simulink model "simulator_prototype_v2"  (R2021b)
(part 11 of 12)

t7145 = ct{1618};
t7148 = ct{1619};
t7149 = ct{1620};
t7150 = ct{1621};
t7152 = ct{1622};
t7153 = ct{1623};
t7156 = ct{1624};
t7157 = ct{1625};
t7159 = ct{1626};
t7160 = ct{1627};
t7163 = ct{1628};
t7164 = ct{1629};
t7166 = ct{1630};
t7167 = ct{1631};
t7168 = ct{1632};
t7169 = ct{1633};
t7171 = ct{1634};
t7172 = ct{1635};
t7175 = ct{1636};
t7176 = ct{1637};
t7179 = ct{1638};
t7181 = ct{1639};
t7185 = ct{1640};
t7186 = ct{1641};
t7195 = ct{1642};
t7196 = ct{1643};
t7200 = ct{1644};
t7201 = ct{1645};
t7202 = ct{1646};
t7203 = ct{1647};
t7204 = ct{1648};
t7209 = ct{1649};
t721 = ct{1650};
t7211 = ct{1651};
t7212 = ct{1652};
t7219 = ct{1653};
t722 = ct{1654};
t7223 = ct{1655};
t7224 = ct{1656};
t7225 = ct{1657};
t7232 = ct{1658};
t7233 = ct{1659};
t7235 = ct{1660};
t724 = ct{1661};
t7240 = ct{1662};
t7242 = ct{1663};
t7245 = ct{1664};
t7246 = ct{1665};
t7250 = ct{1666};
t7252 = ct{1667};
t7253 = ct{1668};
t7254 = ct{1669};
t7255 = ct{1670};
t7257 = ct{1671};
t7259 = ct{1672};
t7266 = ct{1673};
t7268 = ct{1674};
t7277 = ct{1675};
t7278 = ct{1676};
t7282 = ct{1677};
t7284 = ct{1678};
t7285 = ct{1679};
t7286 = ct{1680};
t7287 = ct{1681};
t7288 = ct{1682};
t7290 = ct{1683};
t7292 = ct{1684};
t7293 = ct{1685};
t7295 = ct{1686};
t7296 = ct{1687};
t7297 = ct{1688};
t7298 = ct{1689};
t7299 = ct{1690};
t7300 = ct{1691};
t7301 = ct{1692};
t7302 = ct{1693};
t7303 = ct{1694};
t7304 = ct{1695};
t7305 = ct{1696};
t7306 = ct{1697};
t7307 = ct{1698};
t7308 = ct{1699};
t7309 = ct{1700};
t7311 = ct{1701};
t7313 = ct{1702};
t7316 = ct{1703};
t7317 = ct{1704};
t7325 = ct{1705};
t7326 = ct{1706};
t7331 = ct{1707};
t7333 = ct{1708};
t7334 = ct{1709};
t7336 = ct{1710};
t7337 = ct{1711};
t7339 = ct{1712};
t7340 = ct{1713};
t7342 = ct{1714};
t7343 = ct{1715};
t7345 = ct{1716};
t7346 = ct{1717};
t7347 = ct{1718};
t7349 = ct{1719};
t7351 = ct{1720};
t7353 = ct{1721};
t7354 = ct{1722};
t7359 = ct{1723};
t7360 = ct{1724};
t7361 = ct{1725};
t7362 = ct{1726};
t7363 = ct{1727};
t7371 = ct{1728};
t7372 = ct{1729};
t7375 = ct{1730};
t7381 = ct{1731};
t7382 = ct{1732};
t7384 = ct{1733};
t7386 = ct{1734};
t7388 = ct{1735};
t7394 = ct{1736};
t7404 = ct{1737};
t7405 = ct{1738};
t7407 = ct{1739};
t7411 = ct{1740};
t7412 = ct{1741};
t7416 = ct{1742};
t7417 = ct{1743};
t7418 = ct{1744};
t7419 = ct{1745};
t7429 = ct{1746};
t7430 = ct{1747};
t7431 = ct{1748};
t7432 = ct{1749};
t7433 = ct{1750};
t7440 = ct{1751};
t7443 = ct{1752};
t7444 = ct{1753};
t7445 = ct{1754};
t7446 = ct{1755};
t7447 = ct{1756};
t7453 = ct{1757};
t7459 = ct{1758};
t7461 = ct{1759};
t7478 = ct{1760};
t7479 = ct{1761};
t7482 = ct{1762};
t749 = ct{1763};
t7505 = ct{1764};
t7508 = ct{1765};
t7510 = ct{1766};
t7516 = ct{1767};
t7518 = ct{1768};
t7519 = ct{1769};
t7520 = ct{1770};
t7521 = ct{1771};
t7522 = ct{1772};
t7523 = ct{1773};
t7524 = ct{1774};
t7530 = ct{1775};
t7534 = ct{1776};
t7539 = ct{1777};
t7540 = ct{1778};
t7549 = ct{1779};
t7550 = ct{1780};
t7563 = ct{1781};
t7565 = ct{1782};
t7566 = ct{1783};
t7575 = ct{1784};
t7576 = ct{1785};
t7579 = ct{1786};
t7580 = ct{1787};
t7583 = ct{1788};
t7584 = ct{1789};
t7586 = ct{1790};
t7590 = ct{1791};
t7591 = ct{1792};
t7597 = ct{1793};
t7600 = ct{1794};
t7602 = ct{1795};
t7604 = ct{1796};
t7605 = ct{1797};
t7606 = ct{1798};
t7607 = ct{1799};
t7610 = ct{1800};
t7611 = ct{1801};
t7612 = ct{1802};
t7613 = ct{1803};
t7615 = ct{1804};
t762 = ct{1805};
t7621 = ct{1806};
t7622 = ct{1807};
t7623 = ct{1808};
t7624 = ct{1809};
t7631 = ct{1810};
t7632 = ct{1811};
t7633 = ct{1812};
t7635 = ct{1813};
t7637 = ct{1814};
t7638 = ct{1815};
t7652 = ct{1816};
t7655 = ct{1817};
t7658 = ct{1818};
t7659 = ct{1819};
t7664 = ct{1820};
t7665 = ct{1821};
t7666 = ct{1822};
t7676 = ct{1823};
t768 = ct{1824};
t7680 = ct{1825};
t7682 = ct{1826};
t7683 = ct{1827};
t7684 = ct{1828};
t7686 = ct{1829};
t7689 = ct{1830};
t7691 = ct{1831};
t7692 = ct{1832};
t7698 = ct{1833};
t7699 = ct{1834};
t7703 = ct{1835};
t7710 = ct{1836};
t7730 = ct{1837};
t7731 = ct{1838};
t7732 = ct{1839};
t7733 = ct{1840};
t7734 = ct{1841};
t7735 = ct{1842};
t7736 = ct{1843};
t7738 = ct{1844};
t7741 = ct{1845};
t7745 = ct{1846};
t7746 = ct{1847};
t7748 = ct{1848};
t7749 = ct{1849};
t7751 = ct{1850};
t7754 = ct{1851};
t7757 = ct{1852};
t7759 = ct{1853};
t7762 = ct{1854};
t7765 = ct{1855};
t7766 = ct{1856};
t7768 = ct{1857};
t777 = ct{1858};
t7770 = ct{1859};
t7771 = ct{1860};
t7772 = ct{1861};
t7774 = ct{1862};
t7775 = ct{1863};
t7778 = ct{1864};
t7780 = ct{1865};
t7781 = ct{1866};
t7782 = ct{1867};
t7784 = ct{1868};
t7787 = ct{1869};
t7790 = ct{1870};
t7791 = ct{1871};
t7792 = ct{1872};
t7794 = ct{1873};
t7795 = ct{1874};
t7803 = ct{1875};
t7804 = ct{1876};
t7805 = ct{1877};
t7806 = ct{1878};
t7811 = ct{1879};
t7812 = ct{1880};
t7813 = ct{1881};
t7814 = ct{1882};
t7815 = ct{1883};
t7816 = ct{1884};
t7819 = ct{1885};
t7820 = ct{1886};
t7821 = ct{1887};
t7823 = ct{1888};
t7824 = ct{1889};
t7826 = ct{1890};
t7828 = ct{1891};
t7830 = ct{1892};
t7841 = ct{1893};
t7843 = ct{1894};
t7844 = ct{1895};
t7853 = ct{1896};
t7854 = ct{1897};
t7856 = ct{1898};
t7868 = ct{1899};
t7876 = ct{1900};
t7879 = ct{1901};
t7882 = ct{1902};
t7886 = ct{1903};
t7891 = ct{1904};
t7892 = ct{1905};
t7893 = ct{1906};
t7895 = ct{1907};
t7897 = ct{1908};
t7899 = ct{1909};
t7900 = ct{1910};
t7902 = ct{1911};
t7909 = ct{1912};
t792 = ct{1913};
t7922 = ct{1914};
t7923 = ct{1915};
t7924 = ct{1916};
t7925 = ct{1917};
t7926 = ct{1918};
t7927 = ct{1919};
t7928 = ct{1920};
t7929 = ct{1921};
t793 = ct{1922};
t7930 = ct{1923};
t7931 = ct{1924};
t7933 = ct{1925};
t7934 = ct{1926};
t7952 = ct{1927};
t7953 = ct{1928};
t7954 = ct{1929};
t7967 = ct{1930};
t7968 = ct{1931};
t7969 = ct{1932};
t7971 = ct{1933};
t7973 = ct{1934};
t7975 = ct{1935};
t7976 = ct{1936};
t7989 = ct{1937};
t7990 = ct{1938};
t7991 = ct{1939};
t7992 = ct{1940};
t801 = ct{1941};
t802 = ct{1942};
t808 = ct{1943};
t813 = ct{1944};
t819 = ct{1945};
t821 = ct{1946};
t850 = ct{1947};
t855 = ct{1948};
t874 = ct{1949};
t878 = ct{1950};
t941 = ct{1951};
t948 = ct{1952};
t951 = ct{1953};
t7243 = t6515.*t6606;
t7247 = -t7246;
t7251 = t6564.*t6566;
t7258 = t6515.*t6696;
t7262 = t6566.*t6631;
t7267 = -t7266;
t7318 = t5432+t6552+t6556;
t7332 = -t7331;
t7335 = -t7333;
t7341 = t5526+t6677+t6686;
t7352 = t5624+t6714+t6716;
t7385 = -t6564.*(t4874+t5148-t5704-t6318);
t7389 = t3882.*t7362;
t7390 = -t7363.*(-t1901+t3122+t3270);
t7391 = t3942.*t7362;
t7395 = t3967.*t7363;
t7398 = t5033+t5301+t6320+t7093;
t7399 = -t6696.*(t4786+t5069-t5665-t6291);
t7400 = t6696.*(t4786+t5069-t5665-t6291);
t7401 = t4080.*t7362;
t7403 = -t7363.*(t951+t16.*(-t1881+t3121+t3269));
t7408 = -t6631.*(t4874+t5148-t5704-t6318);
t7409 = t6631.*(t4874+t5148-t5704-t6318);
t7422 = t4780.*t7362;
t7423 = -t7363.*(t17.*((t237.*(t42-t43))./9.007199254740992e+15+t21.*(-t1881+t3121+t3269))+t22.*(-t1901+t3122+t3270));
t7424 = t4822.*t7362;
et371 = -t2306-t2317+t3144+t3147+t35.*t941.*t948.*(t850-t874).*3.775747223193135e-1;
et372 = t36.*t941.*t948.*(t850-t874).*2.244797987218524e-1;
t7426 = -t7363.*(et371+et372);
t7436 = t3481.*t7416;
t7438 = -t17.*t7416.*(t1861-t3214);
t7439 = t17.*t7416.*(t1861-t3214);
t7441 = t3484.*t7417;
t7442 = t17.*t3483.*t7417;
t7448 = t3882.*t7416;
t7450 = -t7417.*(-t1901+t3122+t3270);
t7451 = t7417.*(-t1901+t3122+t3270);
t7456 = t4080.*t7416;
t7457 = -t7417.*(t951+t16.*(-t1881+t3121+t3269));
t7458 = t7417.*(t951+t16.*(-t1881+t3121+t3269));
t7462 = t3481.*t7440;
t7464 = -t17.*t7440.*(t1861-t3214);
t7465 = t3484.*t7443;
t7466 = t17.*t3483.*t7443;
t7474 = t3942.*t7440;
t7476 = t3967.*t7443;
t7483 = -t7482;
t7484 = t7482./2.0;
t7486 = t4780.*t7416;
t7487 = -t7417.*(t17.*((t237.*(t42-t43))./9.007199254740992e+15+t21.*(-t1881+t3121+t3269))+t22.*(-t1901+t3122+t3270));
t7488 = t4822.*t7416;
t7490 = t5787+t6969+t6970;
et373 = -t2306-t2317+t3144+t3147+t35.*t941.*t948.*(t850-t874).*3.775747223193135e-1;
et374 = t36.*t941.*t948.*(t850-t874).*2.244797987218524e-1;
t7491 = -t7417.*(et373+et374);
t7511 = t5895.*t7354;
t7513 = t5898.*t7354;
t7525 = t5895.*t7372;
t7527 = t5898.*t7372;
t7541 = t3481.*t7539;
t7543 = -t17.*t7539.*(t1861-t3214);
t7544 = t17.*t7539.*(t1861-t3214);
t7545 = t3484.*t7540;
t7546 = t17.*t3483.*t7540;
t7551 = -t7550;
t7554 = t3882.*t7539;
t7557 = -t7540.*(-t1901+t3122+t3270);
t7558 = t3942.*t7539;
t7559 = t3967.*t7540;
t7560 = t4080.*t7539;
t7562 = -t7540.*(t951+t16.*(-t1881+t3121+t3269));
t7568 = t4780.*t7539;
t7569 = -t7540.*(t17.*((t237.*(t42-t43))./9.007199254740992e+15+t21.*(-t1881+t3121+t3269))+t22.*(-t1901+t3122+t3270));
t7570 = t4822.*t7539;
et375 = -t2306-t2317+t3144+t3147+t35.*t941.*t948.*(t850-t874).*3.775747223193135e-1;
et376 = t36.*t941.*t948.*(t850-t874).*2.244797987218524e-1;
t7572 = -t7540.*(et375+et376);
t7581 = t6606.*t7354;
t7585 = -t6564.*(t4983-t5225-t6233+t7058);
t7587 = t6696.*t7354;
t7592 = -t6631.*(t4983-t5225-t6233+t7058);
t7593 = t6631.*(t4983-t5225-t6233+t7058);
t7594 = t6606.*t7372;
t7601 = t6696.*t7372;
t7614 = -t7613;
t7627 = t50.*t189.*(t5436+t5438+t6119+t6122+t6536+t6538).*(-9.543032792050485e-17);
t7628 = -t2297.*(t5436+t5438+t6119+t6122+t6536+t6538);
t7629 = t2297.*(t5436+t5438+t6119+t6122+t6536+t6538);
t7630 = -t3047.*(t5436+t5438+t6119+t6122+t6536+t6538);
t7634 = t5184+t5400+t6299+t6301+t6540+t6542;
t7636 = t6678+t6679+t6680+t6687;
t7644 = t6710+t6711+t6713+t6717;
t7651 = t6737+t6738+t6739+t6744;
t7653 = -t7652;
t7654 = t6743+t6746+t6748+t6750;
t7656 = -t7655;
t7662 = -t3210.*(-t6743+t6747+t6510.*(t3544-t4013)+t6512.*(t3544-t4013));
t7669 = -t3483.*(-t6743+t6747+t6510.*(t3544-t4013)+t6512.*(t3544-t4013));
t7673 = -t3877.*(-t6743+t6747+t6510.*(t3544-t4013)+t6512.*(t3544-t4013));
t7675 = -t3957.*(-t6743+t6747+t6510.*(t3544-t4013)+t6512.*(t3544-t4013));
t7678 = t5356+t5513+t6471+t6472+t6669+t6672;
t7679 = t5358+t5512+t6474+t6475+t6673+t6674;
t7681 = t3209.*t7676;
t7687 = -t7676.*(t1861-t3214);
t7688 = t7676.*(t1861-t3214);
t7690 = t6821+t6823+t6824+t6825;
t7693 = t5365+t5586+t6476+t6479+t6695+t6700;
t7697 = -t7676.*(t2674-t2676+t3022-t3027);
t7702 = t3946.*t7676;
t7705 = t3210.*t7691;
t7708 = t3483.*t7691;
t7709 = t6837+t6841+t6842+t6843;
t7712 = t3877.*t7691;
t7715 = t3957.*t7691;
t7718 = t3210.*t7710;
t7722 = t3483.*t7710;
t7727 = t3877.*t7710;
t7729 = t3957.*t7710;
t7737 = -t7736;
t7740 = t5745+t5749+t6482+t6483+t6761+t6762;
t7742 = t5515+t6054+t6150+t6154+t6957+t6962;
t7752 = t5581+t5714+t6596+t6597+t6799+t6800;
t7753 = t5583+t5716+t6598+t6599+t6801+t6803;
t7755 = t3210.*t7751;
t7760 = t3483.*t7751;
t7769 = t3877.*t7751;
t7773 = t3957.*t7751;
t7783 = t7071+t7074+t7076+t7077;
t7788 = t7.*t7787;
t7798 = t5503+t6048+t6656+t6659+t7223+t7225;
t7817 = t5636+t6190+t6779+t6780+t7252+t7253;
t7818 = t5635+t6194+t6781+t6783+t7254+t7255;
t7822 = -t7821;
t7825 = -t7824;
t7831 = t5717+t5718+t5733+t5735+t5963+t5968+t5972+t5973+t6338+t6342+t6351+t6353;
t7837 = t50.*t189.*(t5762-t6289-t6936+t6938+t7266-t7268).*(-9.543032792050485e-17);
t7838 = -t2297.*(t5762-t6289-t6936+t6938+t7266-t7268);
t7839 = -t3047.*(t5762-t6289-t6936+t6938+t7266-t7268);
t7842 = -t7841;
t7845 = -t7844;
t7846 = t5816+t6404+t7019+t7022+t7284+t7285;
t7847 = t5815+t6403+t7023+t7024+t7286+t7287;
t7855 = -t7854;
t7864 = t5414+t6546+t6547+t6577+t7386+t7388;
t7869 = t3128+t3189+t3190+t3200+t3455+t3465+t3470+t4291+t4292+t4362+t4363+t5534+t5538+t5658+t5663+t5764+t5845+t5851+t5945+t5949+t6374+t6380+t6422+t6428;
t7870 = t3128+t3189+t3190+t3200+t3455+t3465+t3470+t4291+t4292+t4362+t4363+t5532+t5537+t5660+t5664+t5764+t5842+t5847+t5947+t5952+t6372+t6377+t6424+t6430;
t7872 = t3128+t3189+t3190+t3200+t3455+t3465+t3470+t4291+t4292+t4362+t4363+t5534+t5538+t5660+t5664+t5764+t5845+t5851+t5947+t5952+t6374+t6380+t6424+t6430;
t7875 = t5883+t6664+t7000+t7001+t7316+t7317;
t7881 = t5622+t5629+t5864+t5865+t5917+t5920+t6218+t6227+t6453+t6459+t6933+t6934;
t7883 = t5622+t5629+t5864+t5865+t5918+t5922+t6222+t6230+t6453+t6459+t6933+t6934;
t7894 = t3210.*t7891;
t7896 = t3483.*t7891;
t7898 = t3877.*t7891;
t7901 = -t7900;
t7903 = t5521+t6667+t6668+t6703+t7429+t7430;
t7908 = t5831+t6707+t6950+t6951+t7418+t7419;
t7911 = t3210.*t7909;
t7914 = t3483.*t7909;
t7919 = t3877.*t7909;
t7921 = t3957.*t7909;
t7935 = t3209.*t7933;
t7936 = t3210.*t7934;
t7938 = -t7933.*(t1861-t3214);
t7939 = t7933.*(t1861-t3214);
t7940 = t3483.*t7934;
t7942 = -t7933.*(t2674-t2676+t3022-t3027);
t7943 = t3877.*t7934;
t7946 = t3946.*t7933;
t7948 = t3957.*t7934;
t7949 = t4680+t4682+t4823+t4826+t5861+t5862+t5912+t5913+t6251+t6252+t6296+t6298+t6729+t6730+t6734+t6736;
t7951 = t2990+t2991+t3054+t3056+t4742+t4772+t4829+t4842+t5855+t5857+t5868+t5871+t6245+t6249+t6282+t6286+t6725+t6728+t6731+t6733;
t7955 = t5771+t6959+t6960+t7087+t7563+t7565;
t7963 = t5203+t5204+t5523+t5525+t5706+t5709+t5779+t5782+t5846+t5850+t5887+t5893+t6235+t6240+t6451+t6452+t6944+t6953;
t7964 = t5203+t5204+t5523+t5525+t5708+t5712+t5779+t5782+t5846+t5850+t5889+t5896+t6239+t6242+t6451+t6452+t6944+t6953;
t7966 = t6047+t7103+t7133+t7135+t7575+t7576;
t7970 = t3210.*t7967;
t7972 = t3483.*t7967;
t7974 = t3877.*t7967;
t7977 = t3957.*t7967;
t7981 = t5563+t5593+t5596+t5820+t5823+t5837+t5838+t6098+t6109+t6360+t6361+t6362+t6795+t7680;
t7982 = t5563+t5593+t5596+t5821+t5825+t5837+t5838+t6099+t6111+t6360+t6361+t6362+t6795+t7680;
t7998 = t5195+t5196+t5367+t5505+t5507+t5559+t5566+t5585+t5808+t5811+t5832+t5833+t5997+t6020+t6114+t6117+t6124+t6348+t6477+t6478+t6534+t6697+t6698+t6777+t7233;
t7999 = t5195+t5196+t5367+t5505+t5507+t5561+t5575+t5585+t5809+t5813+t5832+t5833+t5997+t6020+t6116+t6118+t6124+t6348+t6477+t6478+t6534+t6697+t6698+t6777+t7233;
t8019 = t5361+t5362+t5720+t5721+t5725+t5726+t5727+t5730+t5907+t5910+t5930+t5932+t5959+t5964+t6051+t6053+t6139+t6142+t6199+t6200+t6328+t6335+t6366+t6367+t6441+t6445+t6495+t6500+t6924+t6925+t6979+t6983+t7209+t7212;
t8020 = t5361+t5362+t5720+t5721+t5725+t5726+t5728+t5731+t5908+t5914+t5930+t5932+t5960+t5966+t6051+t6053+t6141+t6143+t6199+t6200+t6333+t6337+t6366+t6367+t6441+t6445+t6496+t6502+t6924+t6925+t6979+t6983+t7209+t7212;
t6204 = t3901.*t5790.*(t1513+t1879+t2598+t2820+t2834+t3117+t3118).*(-7.26735e-3);
t6723 = t5790.*t5895;
t6724 = t5790.*t5898;
t6852 = -t6851;
t6859 = -t6858;
t6895 = -t6894;
t6912 = -t6911;
t6941 = -t6940;
t6977 = -t6976;
t6995 = -t6994;
t7005 = -t7004;
t7007 = -t7006;
t7034 = -t7033;
t7048 = -t7047;
t7067 = -t7066;
t7070 = -t7069;
t7088 = -t7086;
t7117 = -t7116;
t7137 = t5790.*t6606;
t7144 = -t7143;
t7146 = -t7145;
t7154 = -t7153;
t7161 = t5790.*t6696;
t7165 = -t7164;
t7173 = -t7172;
t7319 = t188.*t7318.*8.595599785252598e-1;
t7321 = t2338.*t7318;
t7322 = t2994.*t7318;
t7324 = -t7318.*(t1456-t2355);
t7355 = t2307.*t7352;
t7356 = t17.*t2297.*t7352;
t7357 = -t7352.*(t1456-t2355);
t7392 = -t7391;
t7396 = -t7395;
t7402 = -t7401;
t7425 = -t7424;
t7437 = -t7436;
t7449 = -t7448;
t7463 = -t7462;
t7467 = -t7466;
t7475 = -t7474;
t7477 = -t7476;
t7480 = -t3877.*t7398.*(t1488+t1874+t2519+t2740+t2747+t3096+t3097);
t7485 = -t7484;
t7489 = -t7488;
t7492 = t188.*t7490.*8.595599785252598e-1;
t7494 = t2307.*t7490;
t7495 = t17.*t2297.*t7490;
t7496 = t2338.*t7490;
t7498 = t2994.*t7490;
t7500 = -t7490.*(t1456-t2355);
t7501 = t7490.*(t1456-t2355);
t7512 = -t7511;
t7514 = -t7513;
t7526 = -t7525;
t7528 = -t7527;
t7537 = t5800.*t7398;
t7538 = t5801.*t7398;
t7542 = -t7541;
t7561 = -t7560;
t7571 = -t7570;
t7582 = -t7581;
t7588 = -t7587;
t7598 = t6564.*t7398;
t7608 = t6631.*t7398;
t7616 = t6550+t6551+t6553+t6554;
t7639 = t50.*t189.*t7636.*9.543032792050485e-17;
t7641 = t2297.*t7636;
t7642 = t3047.*t7636;
t7645 = t50.*t189.*t7644.*9.543032792050485e-17;
t7646 = t2297.*t7644;
t7647 = t3047.*t7644;
t7660 = t3209.*t7651;
t7667 = -t7651.*(t1861-t3214);
t7668 = t7651.*(t1861-t3214);
t7671 = -t7651.*(t2674-t2676+t3022-t3027);
t7672 = t7651.*(t2674-t2676+t3022-t3027);
t7674 = t3946.*t7651;
t7694 = t50.*t189.*t7693.*9.543032792050485e-17;
t7696 = t2297.*t7693;
t7700 = t3047.*t7693;
t7704 = t3209.*t7690;
t7706 = -t7690.*(t1861-t3214);
t7707 = t7690.*(t1861-t3214);
t7711 = -t7690.*(t2674-t2676+t3022-t3027);
t7713 = -t7712;
t7714 = t3946.*t7690;
t7716 = t3209.*t7709;
t7719 = -t7718;
t7720 = -t7709.*(t1861-t3214);
t7721 = t7709.*(t1861-t3214);
t7725 = -t7709.*(t2674-t2676+t3022-t3027);
t7726 = t7709.*(t2674-t2676+t3022-t3027);
t7728 = t3946.*t7709;
t7756 = -t7755;
t7761 = t3209.*t7752;
t7763 = -t7752.*(t1861-t3214);
t7764 = t7752.*(t1861-t3214);
t7776 = -t7752.*(t2674-t2676+t3022-t3027);
t7777 = t7752.*(t2674-t2676+t3022-t3027);
t7779 = t3946.*t7752;
t7789 = t7788./2.0;
t7796 = t5904+t5906+t6129+t6132+t7644;
t7797 = t5904+t5906+t6130+t6134+t7644;
t7799 = t50.*t189.*t7798.*9.543032792050485e-17;
t7801 = t2297.*t7798;
t7802 = t3047.*t7798;
t7836 = t5763+t6289+t6936+t6939+t7267+t7268;
t7848 = t3209.*t7846;
t7849 = t3210.*t7847;
t7850 = -t7846.*(t1861-t3214);
t7851 = t3483.*t7847;
t7857 = -t7846.*(t2674-t2676+t3022-t3027);
t7858 = t7846.*(t2674-t2676+t3022-t3027);
t7859 = t3877.*t7847;
t7860 = t3946.*t7846;
t7861 = t3957.*t7847;
t7865 = t50.*t189.*t7864.*9.543032792050485e-17;
t7867 = t2297.*t7864;
t7871 = t3047.*t7864;
t7877 = t3210.*t7875;
t7880 = t3483.*t7875;
t7884 = t3877.*t7875;
t7887 = t3957.*t7875;
t7888 = t6645+t6653+t6682+t6683+t6684+t6685+t7094+t7095;
t7889 = t6649+t6655+t6682+t6683+t6684+t6685+t7094+t7095;
t7904 = t50.*t189.*t7903.*9.543032792050485e-17;
t7906 = t2297.*t7903;
t7907 = t3047.*t7903;
t7910 = t3209.*t7908;
t7912 = -t7908.*(t1861-t3214);
t7913 = t7908.*(t1861-t3214);
t7917 = -t7908.*(t2674-t2676+t3022-t3027);
t7918 = t7908.*(t2674-t2676+t3022-t3027);
t7920 = t3946.*t7908;
t7937 = -t7936;
t7941 = -t7940;
t7944 = t5770+t6019+t6414+t6415+t6876+t6880+t6884+t6891+t7053+t7063;
t7945 = t5770+t6019+t6414+t6415+t6878+t6882+t6884+t6891+t7053+t7063;
t7947 = -t7946;
t7956 = t50.*t189.*t7955.*9.543032792050485e-17;
t7958 = t2297.*t7955;
t7959 = t3047.*t7955;
t7993 = t5372+t5436+t5438+t6079+t6080+t6084+t6119+t6122+t6160+t6166+t6505+t6521+t6528+t6536+t6538+t6559+t6562+t7010+t7017;
t7994 = t5372+t5436+t5438+t6079+t6080+t6084+t6119+t6122+t6161+t6168+t6505+t6521+t6528+t6536+t6538+t6560+t6563+t7010+t7017;
t7995 = t5288+t5514+t5793+t5818+t5819+t6034+t6144+t6155+t6406+t6407+t6900+t6902+t7050+t7052+t7308+t7311;
t7996 = t5288+t5514+t5793+t5818+t5819+t6034+t6144+t6155+t6406+t6407+t6900+t6902+t7050+t7052+t7309+t7313;
t8012 = t4661+t4683+t5306+t5308+t5480+t5481+t5483+t5484+t5670+t5671+t5674+t5675+t7664+t7666+t7766+t7769;
t8033 = t4413+t4579+t5380+t5399+t6543+t6544+t6658+t6663+t7105+t7106+t7109+t7110+t7549+t7604+t7605+t7627+t7681+t7682;
t8035 = t5055+t5666+t5693+t6058+t6489+t6491+t6988+t6989+t7039+t7041+t7242+t7243+t7516+t7519+t7853+t7864;
t8036 = t5055+t5666+t5693+t6058+t6490+t6492+t6988+t6989+t7039+t7041+t7242+t7243+t7518+t7520+t7853+t7864;
t8038 = t5328+t5407+t6958+t6963+t7245+t7247+t7815+t7816+t7825+t7826;
t7320 = -t7319;
t7323 = -t7322;
t7493 = -t7492;
t7497 = -t7495;
t7499 = -t7498;
t7609 = -t7608;
t7617 = t50.*t189.*t7616.*9.543032792050485e-17;
t7618 = t2297.*t7616;
t7620 = t3047.*t7616;
t7640 = -t7639;
t7643 = -t7642;
t7648 = -t7647;
t7695 = -t7694;
t7701 = -t7700;
t7717 = -t7716;
t7785 = t7163+t7165+t7166+t7167;
t7786 = t7168+t7169+t7171+t7173;
t7800 = -t7799;
t7832 = t5994+t6688+t6694+t6773+t6775+t7030+t7034;
t7833 = t5994+t6690+t6699+t6773+t6775+t7030+t7034;
t7834 = t6004+t6720+t6723+t6788+t6792+t7089+t7090;
t7835 = t6004+t6722+t6724+t6788+t6792+t7089+t7090;
t7852 = -t7851;
t7862 = t6548+t6555+t6557+t6558+t6613+t6615+t7040+t7048;
t7863 = t6548+t6555+t6557+t6558+t6614+t6616+t7040+t7048;
t7866 = -t7865;
t7873 = -t7871;
t7885 = -t7884;
t7905 = -t7904;
t7932 = t6584+t6585+t6603+t6609+t7150+t7154+t7159+t7160;
t7950 = t6752+t6754+t6764+t6765+t7139+t7140+t7142+t7146;
t7957 = -t7956;
t7960 = -t7959;
t7965 = t5339+t5342+t5700+t5701+t5702+t5703+t7726+t7727;
t7979 = t5760+t6010+t6102+t6107+t6356+t6365+t6388+t6392+t6622+t6627+t6854+t6857+t7003+t7007;
t7980 = t5760+t6010+t6105+t6112+t6356+t6365+t6388+t6392+t6624+t6629+t6854+t6857+t7003+t7007;
t7983 = t5344+t5494+t6178+t6188+t6905+t6907+t7672+t7673;
t7986 = t5243+t5384+t6232+t6236+t6973+t6977+t7711+t7713;
t7987 = t4963+t5685+t5687+t5786+t6028+t6317+t6322+t6375+t6378+t6601+t6610+t6864+t6865+t6870+t6871+t6991+t6995;
t7988 = t4963+t5685+t5687+t5786+t6028+t6317+t6322+t6375+t6378+t6605+t6612+t6865+t6866+t6870+t6872+t6991+t6995;
t7997 = t7858+t7859;
t8002 = t5254+t5383+t6202+t6204+t6926+t6931+t7646+t7721+t7722;
t8006 = t5317+t5320+t7152+t7156+t7157+t7161+t7641+t7707+t7708;
t8007 = t7060+t7067+t7303+t7306+t7792+t7798;
t8008 = t7060+t7067+t7305+t7307+t7792+t7798;
t8009 = t5289+t5516+t5900+t5924+t5925+t6169+t6293+t6295+t6937+t6942+t7201+t7203+t7259+t7262+t7522+t7526;
t8010 = t5289+t5516+t5900+t5924+t5925+t6169+t6293+t6295+t6937+t6942+t7201+t7203+t7259+t7262+t7524+t7528;
t8011 = t7324+t7392+t7396+t7630+t7702+t7703;
t8014 = t7357+t7475+t7477+t7692+t7772+t7773;
t8015 = t7837+t7848+t7849;
t8016 = t4496+t4652+t5227+t5444+t5890+t5891+t6103+t6106+t6484+t6486+t6886+t6895+t7612+t7614+t7697+t7699;
t8017 = t7842+t7876+t7877;
t8018 = t7843+t7879+t7880;
t8021 = t4432+t5198+t5250+t5396+t5397+t5499+t5866+t5870+t5875+t6075+t6076+t6156+t6238+t6241+t6436+t6439+t6913+t6916+t6917+t6919+t7195+t7196+t7250+t7251+t7508+t7512;
t8022 = t4432+t5198+t5250+t5396+t5397+t5499+t5866+t5870+t5875+t6075+t6076+t6156+t6238+t6241+t6437+t6442+t6913+t6916+t6917+t6919+t7195+t7196+t7250+t7251+t7510+t7514;
t8023 = t7257+t7258+t7530+t7537+t7899+t7903;
t8024 = t7257+t7258+t7534+t7538+t7899+t7903;
t8025 = t7345+t7439+t7442+t7802+t7828+t7830;
t8026 = t4221+t4244+t4664+t4703+t5245+t5246+t5247+t5248+t5346+t5349+t5433+t5434+t5440+t5441+t5678+t5679+t5681+t5682+t7296+t7297+t7777+t7778+t7781+t7782;
t8027 = t5316+t5695+t7114+t7117+t7175+t7176+t7551+t7607+t7610+t7629+t7688+t7689;
t8028 = t7571+t7572+t7973+t7974;
t8029 = t5347+t5524+t6438+t6444+t6910+t6912+t7623+t7658+t7659+t7686+t7759+t7760;
t8032 = t4615+t4642+t5252+t5428+t5791+t5792+t6090+t6093+t6247+t6253+t6839+t6852+t7622+t7653+t7656+t7684+t7754+t7756;
t8034 = t7501+t7558+t7559+t7845+t7886+t7887;
t8039 = t7351+t7486+t7487+t7907+t7947+t7948;
t8042 = t7496+t7561+t7562+t7958+t7971+t7972;
t8045 = t5337+t5405+t6920+t6921+t7232+t7235+t7355+t7375+t7459+t7461+t7463+t7465+t7696+t7738+t7764+t7765+t7774+t7775;
t8046 = t5389+t5492+t6984+t6985+t7099+t7100+t7431+t7433+t7479+t7480+t7489+t7491+t7928+t7930+t7942+t7943;
t8047 = t5377+t5379+t7335+t7346+t7382+t7384+t7394+t7400+t7407+t7409+t7437+t7441+t7795+t7801+t7813+t7814+t7822+t7823;
t8048 = t4911+t5007+t5488+t5580+t6206+t6209+t6507+t6511+t6691+t6692+t6935+t6941+t7079+t7088+t7107+t7108+t7360+t7361+t7425+t7426+t7445+t7447+t7733+t7734+t7897+t7898+t7918+t7919;
t8049 = t5517+t5552+t7301+t7321+t7339+t7340+t7402+t7403+t7590+t7591+t7593+t7594+t7856+t7867+t7895+t7896+t7913+t7914;
t7619 = -t7618;
t7978 = t7620+t7674+t7675;
t7984 = t7643+t7714+t7715;
t7985 = t7648+t7728+t7729;
t8000 = t7882+t7885;
t8001 = t5350+t5493+t6157+t6159+t6868+t6874+t7645+t7717+t7719;
t8003 = t5496+t5500+t7111+t7112+t7113+t7115+t7617+t7660+t7662;
t8005 = t5381+t5411+t7123+t7126+t7148+t7149+t7640+t7704+t7705;
t8013 = t7356+t7464+t7467+t7701+t7779+t7780;
t8030 = t7494+t7542+t7545+t7838+t7850+t7852;
t8031 = t7497+t7544+t7546+t7839+t7860+t7861;
t8037 = t7323+t7422+t7423+t7873+t7920+t7921;
t8040 = t4647+t4931+t5498+t5631+t6219+t6221+t6339+t6341+t6427+t6432+t6856+t6859+t7240+t7277+t7278+t7695+t7737+t7761+t7762+t7768+t7770;
t8041 = t7493+t7554+t7557+t7957+t7969+t7970;
t8043 = t7499+t7568+t7569+t7960+t7976+t7977;
t8044 = t5490+t5694+t7185+t7186+t7381+t7385+t7794+t7800+t7811+t7812+t7819+t7820;
t8050 = t5518+t5531+t7332+t7343+t7404+t7405+t7449+t7451+t7586+t7588+t7597+t7598+t7901+t7905+t7923+t7924+t7935+t7937;
t8051 = t5482+t5487+t7334+t7347+t7411+t7412+t7456+t7458+t7600+t7601+t7606+t7609+t7902+t7906+t7925+t7926+t7939+t7941;
t8052 = t4870+t4871+t5620+t5627+t6810+t6811+t6813+t6892+t6893+t7055+t7056+t7300+t7320+t7336+t7337+t7389+t7390+t7580+t7582+t7584+t7585+t7665+t7730+t7732+t7855+t7866+t7893+t7894+t7910+t7911;
t8004 = t5402+t5403+t7132+t7137+t7141+t7144+t7619+t7668+t7669;
et377 = -t5289-t5516-t5900+t5923-t6169+t6294-t6942+t7200+t7202-t7262+t7521+t7525;
et378 = t4080.*(t4510.*(t2813-t2835+t18.*(t1456-t2355).*1.02e-6+t23.*(t1456-t2355).*9.0e-8)+t4514.*(-t2804+t2838+t3109+t23.*(t1456-t2355).*9.3e-7)+t3132.*(t3235-t3535));
et379 = t6565.*(t4758.*(t1861-t3214)+t2297.*(t642+t643-t667+t674+t1587+t1606+t1608+t1609+t2295+t2671+t2683+t2684-t2695+t3272+t3290-t3296+t3576+t3582+t3588-t3593+t4015+t4016))+t5756.*(t951+t16.*(-t1881+t3121+t3269))+(t1861-t3214).*(t4595+t4658+t5189+t5207-t3468.*(t1005+t26.*(t1941-t3308+t39.*t1022.*(t855-t878).*2.196325630278387e-1))-t3420.*(t1896-t3232));
et380 = t707+t708-t721-t722-t749+t762+t768-t777-t792-t793-t801-t802-t808+t813-t819+t821-t1629+t1637-t1640-t1641-t1659-t1661+t1666+t1667+t1683+t1692+t1705-t1712+t1758+t1759+t1775+t1776+t1973+t1993+t1994+t2023+t2053+t2060-t2089-t2090+t2098+t2099-t14.*t15.*t21.*t50.*t189.*3.670836568391568e-22;
et381 = t16.*t19.*t20.*t50.*t189.*(-3.279367663374749e-19)-t14.*t15.*t17.*t21.*t50.*t189.*7.075931802640439e-19;
et382 = t14.*t17.*t20.*t21.*t50.*t189.*(-1.190170786299927e-18)-t15.*t17.*t19.*t21.*t50.*t189.*1.190170786299927e-18;
et383 = t19.*t20.*t21.*t22.*t50.*t189.*(-3.226512155691387e-19);
et384 = t3563.*1.33637554986e-4+t3693-t3694+t33.*(t1896-t3232).*4.36041e-5;
et385 = t33.*t34.*(t1896-t3232).*7.26350557185e-5;
et386 = -t5204+t5522+t5705+t5775-t5782+t5892+t6234-t6240+t6450+t6949+t3877.*(t3959+t4200-t4287+t4409+t3996.*(t2801-t2850)+t3992.*(t335-t1539-t2831+t2851))+t6807.*(t2674-t2676+t3022-t3027)+(t2674-t2676+t3022-t3027).*(et384+et385).*(t1488+t1874+t2519+t2740+t2747+t3096+t3097)+t3617.*t4324.*(t2674-t2676+t3022-t3027)+t3689.*t5588.*(t2674-t2676+t3022-t3027)+t3313.*t3877.*(-t321+t332+t1196+t1212+t1237+t1238+t2139+t2140+t2159+t2165+t2754+t2814+t2953+t3072+t3405+t3412);
et387 = t3877.*t4134.*(t3410-t3708+t3714+t26.*t50.*t202.*(t46-t47).*8.687615694748404e-39)+t3877.*t5314.*(t1488+t1874+t2519+t2740+t2747+t3096+t3097);
et388 = t3563.*1.33637554986e-4+t3693-t3694+t33.*(t1896-t3232).*4.36041e-5;
et389 = t33.*t34.*(t1896-t3232).*7.26350557185e-5;
et390 = t3563.*1.33637554986e-4+t3693-t3694+t33.*(t1896-t3232).*4.36041e-5;
et391 = t33.*t34.*(t1896-t3232).*7.26350557185e-5;
et392 = t4.*(et386+et387)-t2.*t7868+t6.*t7995-t3.*(t3560+t3790+t3791+t3861+t3862+t4154+t4898-t5534-t5538+t5659+t5662-t5845-t5851+t5946+t5948+t6018+t6379+t6423+t6425+t5799.*(et388+et389))+t7.*(-t5515-t6054+t6147+t6956+t6961+t17.*t3483.*(t4311-t5186+t4541.*(-t2804+t2838+t3109+t23.*(t1456-t2355).*9.3e-7)));
et393 = t5.*(-t4963-t5685-t5687+t5785-t6028-t6317+t6321+t6600+t6608+t6863-t6864+t6869-t6871+t6994+t6561.*(et390+et391)+t3210.*(t3959+t4200-t4287+t4409+t3996.*(t2801-t2850)+t3992.*(t335-t1539-t2831+t2851))+t3209.*(-t4196+t4285+t4582+t3206.*(t1896-t3232)+t3985.*(t2801-t2850)+t27.*t3863.*(t1896-t3232)));
et394 = t5621+t5628+t5919+t6226-t6453-t6459+t6932-t6934+t3782.*t5588.*(t2674-t2676+t3022-t3027)+t3892.*t5884.*(t2674-t2676+t3022-t3027);
et395 = (t3349-t3649+t28.*(t3235-t3535).*1.33637554986e-4+t34.*(t3235-t3535).*7.26350557185e-5).*(t2674-t2676+t3022-t3027).*(t1488+t1874+t2519+t2740+t2747+t3096+t3097)+t3877.*t5321.*(t1488+t1874+t2519+t2740+t2747+t3096+t3097);
et396 = t50.*t189.*(-t4447+t4458+t3385.*(t2813-t2835+t18.*(t1456-t2355).*1.02e-6+t23.*(t1456-t2355).*9.0e-8)+t3386.*(-t2804+t2838+t3109+t23.*(t1456-t2355).*9.3e-7));
et397 = 9.543032792050485e-17;
et398 = t4.*(t7788-t2.*t7992-t3.*t7991+t4.*t8019+t5.*t8021-t6.*(et377+et378+et379))+t3.*(t6.*t7786-t4.*t7831+t2.*t7951-t5.*(t6585+t6603+t6609+t7150+t7154+t7159+t7160-t5539.*(et380+et381+et382+et383))+t3.*(t4679-t4680+t4816+t5859+t5860-t5913+t6248-t6296+t6297+t6727-t6729-t6734+t6735+t5539.*(t410-t5413)+t3847.*(t313-t314-t1108+t1115-t1158-t1159-t2117+t2120+t2122+t2123)+t5151.*(-t321+t332+t1196+t1212+t1237+t1238+t2139+t2140+t2159+t2165+t2754+t2814+t2953+t3072+t3405+t3412)))+t5.*(et392+et393)-t6.*(t7748+t2.*t7803+t3.*t7804-t6.*t7944+t5.*t7979-t4.*(et394+et395));
et399 = t7.*(t7482+t5.*(-t6688-t6694+t6772+t6774+t7033+t6561.*(t3547.*1.33637554986e-4+t4119-t4120+t34.*(t1896-t3232).*7.26350557185e-5)+et396.*et397)-t2.*t7631-t3.*t7632-t4.*t7745+t6.*t7834);
et400 = t6030-t6943-t6945+t3942.*(t4510.*(t2813-t2835+t18.*(t1456-t2355).*1.02e-6+t23.*(t1456-t2355).*9.0e-8)+t4514.*(-t2804+t2838+t3109+t23.*(t1456-t2355).*9.3e-7)+t3132.*(t3235-t3535))+t5489.*(t1456-t2355);
et401 = t3967.*(t4311-t5186+t4541.*(-t2804+t2838+t3109+t23.*(t1456-t2355).*9.3e-7));
et402 = t707+t708-t721-t722-t749+t762+t768-t777-t792-t793-t801-t802-t808+t813-t819+t821-t1629+t1637-t1640-t1641-t1659-t1661+t1666+t1667+t1683+t1692+t1705-t1712+t1758+t1759+t1775+t1776+t1973+t1993+t1994+t2023+t2053+t2060-t2089-t2090+t2098+t2099-t14.*t15.*t21.*t50.*t189.*3.670836568391568e-22;
et403 = t16.*t19.*t20.*t50.*t189.*(-3.279367663374749e-19)-t14.*t15.*t17.*t21.*t50.*t189.*7.075931802640439e-19;
et404 = t14.*t17.*t20.*t21.*t50.*t189.*(-1.190170786299927e-18)-t15.*t17.*t19.*t21.*t50.*t189.*1.190170786299927e-18;
et405 = t19.*t20.*t21.*t22.*t50.*t189.*(-3.226512155691387e-19);
et406 = -t5760+t6009+t6104-t6356+t6387-t6392+t6623+t6628-t6854-t6857+t7006+t5223.*(t350+t366-t1205+t1210-t1217-t1218-t2147+t2152+t2154+t2155-t3395-t3399-t3409-t3716+t3723+t32.*t50.*t202.*(t46-t47).*8.687615694748404e-39)+t4975.*(et402+et403+et404+et405);
et407 = t6561.*(t3349-t3649+t28.*(t3235-t3535).*1.33637554986e-4+t34.*(t3235-t3535).*7.26350557185e-5);
et408 = t707+t708-t721-t722-t749+t762+t768-t777-t792-t793-t801-t802-t808+t813-t819+t821-t1629+t1637-t1640-t1641-t1659-t1661+t1666+t1667+t1683+t1692+t1705-t1712+t1758+t1759+t1775+t1776+t1973+t1993+t1994+t2023+t2053+t2060-t2089-t2090+t2098+t2099-t14.*t15.*t21.*t50.*t189.*3.670836568391568e-22;
et409 = t16.*t19.*t20.*t50.*t189.*(-3.279367663374749e-19)-t14.*t15.*t17.*t21.*t50.*t189.*7.075931802640439e-19;
et410 = t14.*t17.*t20.*t21.*t50.*t189.*(-1.190170786299927e-18)-t15.*t17.*t19.*t21.*t50.*t189.*1.190170786299927e-18;
et411 = t19.*t20.*t21.*t22.*t50.*t189.*(-3.226512155691387e-19);
et412 = t3563.*1.33637554986e-4+t3693-t3694+t33.*(t1896-t3232).*4.36041e-5;
et413 = t33.*t34.*(t1896-t3232).*7.26350557185e-5;
et414 = -t5204+t5522+t5707+t5711+t5775-t5782+t5894+t6237-t6242+t6450+t6949+t3877.*(t3959+t4200-t4287+t4409+t3996.*(t2801-t2850)+t3992.*(t335-t1539-t2831+t2851))+t6807.*(t2674-t2676+t3022-t3027)+(t2674-t2676+t3022-t3027).*(et412+et413).*(t1488+t1874+t2519+t2740+t2747+t3096+t3097)+t3617.*t4324.*(t2674-t2676+t3022-t3027)+t3689.*t5589.*(t2674-t2676+t3022-t3027);
et415 = t3877.*t4134.*(t3410-t3708+t3714+t26.*t50.*t202.*(t46-t47).*8.687615694748404e-39)+t3877.*t5314.*(t1488+t1874+t2519+t2740+t2747+t3096+t3097);
et416 = t3563.*1.33637554986e-4+t3693-t3694+t33.*(t1896-t3232).*4.36041e-5;
et417 = t33.*t34.*(t1896-t3232).*7.26350557185e-5;
et418 = t1288+t1289+t1302+t1303-t1319-t1320+t1336-t1348+t1350+t1351-t1360+t1369-t1378+t1396-t1425+t1435-t2174+t2183-t2187+t2193-t2194-t2195+t2199-t2203-t2215+t2219-t2222-t2223+t2239+t2240-t2256-t2257+t2555+t2556+t2572+t2583-t2605-t2606+t2612+t2613-t2618-t2619+t2651+t2652;
et419 = t24.*t25.*t26.*t50.*t202.*(-3.566935413776081e-21);
et420 = t30.*t31.*t32.*t50.*t202.*(-3.992732227073824e-24);
et421 = t24.*t25.*t32.*t33.*t50.*t202.*(-3.509445006623964e-21);
et422 = t27.*t30.*t31.*t32.*t50.*t202.*(-7.696420262413979e-21);
et423 = t2.*t7870+t3.*t7872+t6.*t7996+t4.*(et414+et415)+t7.*(-t5515-t6054+t6147+t6956+t6961+t17.*t3483.*(t4311-t5186+t4541.*(-t2804+t2838+t3109+t23.*(t1456-t2355).*9.3e-7)));
et424 = t5.*(-t4963-t5685-t5687+t5785-t6028-t6317+t6321+t6604+t6611+t6863-t6866+t6869-t6872+t6994+t6561.*(et416+et417)+t3210.*(t3959+t4200-t4287+t4409+t3996.*(t2801-t2850)+t3992.*(t335-t1539-t2831+t2851))+t3209.*(-t4196+t4285+t4582+t3206.*(t1896-t3232)+t3985.*(t2801-t2850)+t27.*t3863.*(t1896-t3232)))+(t2.*(t6753+t6763-t6765+t7138-t7140-t7142+t7145+t5412.*(et418+et419+et420+et421+et422)))./2.0;
et425 = -t5289-t5516-t5900+t5923-t6169+t6294-t6942+t7200+t7202-t7262+t7523+t7527;
et426 = t4080.*(t4510.*(t2813-t2835+t18.*(t1456-t2355).*1.02e-6+t23.*(t1456-t2355).*9.0e-8)+t4514.*(-t2804+t2838+t3109+t23.*(t1456-t2355).*9.3e-7)+t3132.*(t3235-t3535));
et427 = t6565.*(t4758.*(t1861-t3214)+t2297.*(t642+t643-t667+t674+t1587+t1606+t1608+t1609+t2295+t2671+t2683+t2684-t2695+t3272+t3290-t3296+t3576+t3582+t3588-t3593+t4015+t4016))+t5756.*(t951+t16.*(-t1881+t3121+t3269))+(t1861-t3214).*(t4595+t4658+t5189+t5207-t3468.*(t1005+t26.*(t1941-t3308+t39.*t1022.*(t855-t878).*2.196325630278387e-1))-t3420.*(t1896-t3232));
et428 = t50.*t189.*(-t4447+t4458+t3385.*(t2813-t2835+t18.*(t1456-t2355).*1.02e-6+t23.*(t1456-t2355).*9.0e-8)+t3386.*(-t2804+t2838+t3109+t23.*(t1456-t2355).*9.3e-7));
et429 = 9.543032792050485e-17;
et430 = t5412.*(t350+t366-t1205+t1210-t1217-t1218-t2147+t2152+t2154+t2155-t3395-t3399-t3409-t3716+t3723+t32.*t50.*t202.*(t46-t47).*8.687615694748404e-39);
et431 = -t5426.*(t350+t366-t1205+t1210-t1217-t1218-t2147+t2152+t2154+t2155-t3395-t3399-t3409-t3716+t3723+t32.*t50.*t202.*(t46-t47).*8.687615694748404e-39)+t3850.*t4109-t3866.*t4109+t5092.*t5307-t5150.*t5307+t5413.*t5589-t5437.*t5589+t5797.*t5888-t5800.*t5888-t5796.*t5898+t5798.*t5898;
et432 = t3849.*(t1089-t1104-t1105-t1121-t2117+t2120+t2122+t2123)-t3865.*(t1089-t1104-t1105-t1121-t2117+t2120+t2122+t2123)-t5304.*(t649+t670+t686+t687+t1577+t1578+t1586+t1600+t2303+t2339+t2689+t3030+t3292+t3305)+t5304.*(-t56+t60+t649+t670+t686+t687+t1577+t1578+t1586+t1600+t2303+t2339+t2689+t3030+t3292+t3305);
et433 = t6.*((t2.*t7785)./2.0-t2.*t7805-t3.*t7806-t4.*t7883+t6.*t7945+t7.*(et400+et401)+t5.*(et406+et407))-t2.*((t6.*t7786)./2.0-(t4.*t7831)./2.0+(t2.*t7951)./2.0-(t5.*(t6585+t6603+t6609+t7150+t7154+t7159+t7160-t5539.*(et408+et409+et410+et411)))./2.0+(t3.*(t4679-t4680+t4816+t5859+t5860-t5913+t6248-t6296+t6297+t6727-t6729-t6734+t6735+t5539.*(t410-t5413)+t3847.*(t313-t314-t1108+t1115-t1158-t1159-t2117+t2120+t2122+t2123)+t5151.*(-t321+t332+t1196+t1212+t1237+t1238+t2139+t2140+t2159+t2165+t2754+t2814+t2953+t3072+t3405+t3412)))./2.0)+t5.*(et423+et424);
et434 = t4.*(t7788-t2.*t7990-t3.*t7989+t4.*t8020+t5.*t8022+(t2.*(t5595+t5601-t5617-t5619-t5858+t5873+t5885+t6223+t6229-t6256+t4175.*t5413.*(t2694-t2701+t3036-t3043).*1.08769e-2+t3901.*t5798.*(t1513+t1879+t2598+t2820+t2834+t3117+t3118).*7.26735e-3))./2.0-t6.*(et425+et426+et427));
et435 = t7.*(t7482+t5.*(-t6690-t6699+t6772+t6774+t7033+t6561.*(t3547.*1.33637554986e-4+t4119-t4120+t34.*(t1896-t3232).*7.26350557185e-5)+et428.*et429)-t2.*t7633-t3.*t7635-t4.*t7746+t6.*t7835);
et436 = (t2.*t3.*(et430+et431+et432))./2.0;
et437 = t5031-t7091+t4795.*(t1005+t26.*(t1941-t3308+t39.*t1022.*(t855-t878).*2.196325630278387e-1)).*7.26735e-3;
et438 = t2419.*(t684+t685-t710+t724+t1686-t1690+t1700+t1701+t2371+t2698+t2707-t2716+t2719+t3319-t3327-t3341-t3620+t3622+t3634-t3638+t4076+t4077).*7.26735e-3;
et439 = -t5518-t5531+t7331+t7342-t7405+t7448+t7450+t7587-t7598+t7900+t7904+t7922-t7935+t7936+t6561.*(et437+et438)+t7353.*(t4795.*(t1896-t3232).*7.26735e-3+t2363.*(t684+t685-t710+t724+t1686-t1690+t1700+t1701+t2371+t2698+t2707-t2716+t2719+t3319-t3327-t3341-t3620+t3622+t3634-t3638+t4076+t4077).*7.26735e-3);
et440 = t3882.*(t6767+t6001.*(t1896-t3232)+t3985.*(t3424-t3437+t4552+t4556+t3942.*(t1896-t3232).*5.7e-7+t3946.*(t1896-t3232).*4.0e-8));
et441 = t3210.*(t6179-t6903-t7211+t7282+t7453+t4824.*(t3424-t3437+t4552+t4556+t3942.*(t1896-t3232).*5.7e-7+t3946.*(t1896-t3232).*4.0e-8));
et442 = t5592+t5594+t5822+t5836+t6108+t6389-t6391-t6675-t6676+t7621+t3057.*(t4752+t3942.*(t2694-t2701+t3036-t3043).*1.02e-6)+t5520.*(t1477-t2502)+t3784.*t5426.*(t2694-t2701+t3036-t3043).*1.08769e-2+t3918.*t5798.*(t2694-t2701+t3036-t3043).*7.26735e-3;
et443 = t3901.*t5262.*(t1513+t1879+t2598+t2820+t2834+t3117+t3118).*7.26735e-3;
et444 = t5592+t5594+t5824+t5836+t6110+t6389-t6391-t6675-t6676+t7621+t3057.*(t4752+t3942.*(t2694-t2701+t3036-t3043).*1.02e-6)+t5520.*(t1477-t2502)+t3784.*t5429.*(t2694-t2701+t3036-t3043).*1.08769e-2+t3918.*t5799.*(t2694-t2701+t3036-t3043).*7.26735e-3;
et445 = t3901.*t5262.*(t1513+t1879+t2598+t2820+t2834+t3117+t3118).*7.26735e-3;
et446 = -t2306-t2317+t3144+t3147+t35.*t941.*t948.*(t850-t874).*3.775747223193135e-1;
et447 = t36.*t941.*t948.*(t850-t874).*2.244797987218524e-1;
et448 = t707+t708-t721-t722-t749+t762+t768-t777-t792-t793-t801-t802-t808+t813-t819+t821-t1629+t1637-t1640-t1641-t1659-t1661+t1666+t1667+t1683+t1692+t1705-t1712+t1758+t1759+t1775+t1776+t1973+t1993+t1994+t2023+t2053+t2060-t2089-t2090+t2098+t2099-t14.*t15.*t21.*t50.*t189.*3.670836568391568e-22;
tau_c = ft_17({et398,et399,et433,et434,et435,et436,et439,et440,et441,et442,et443,et444,et445,et446,et447,et448,t1005,t1022,t1196,t1205,t1210,t1212,t1217,t1218,t123,t1237,t1238,t1288,t1289,t1302,t1303,t1319,t1320,t1336,t1348,t1350,t1351,t1360,t1369,t1378,t1396,t14,t140,t1425,t1435,t1456,t1477,t1488,t15,t1513,t1539,t1554,t1577,t1578,t1586,t1587,t16,t1600,t1606,t1608,t1609,t1629,t1637,t1640,t1641,t1659,t1661,t1666,t1667,t1683,t1686,t1690,t1692,t17,t1700,t1701,t1705,t1712,t1758,t1759,t1775,t1776,t18,t1861,t1874,t1879,t188,t1881,t189,t1896,t19,t1901,t1941,t1959,t1973,t1993,t1994,t2,t20,t201,t202,t2023,t2053,t2060,t2089,t2090,t2098,t2099,t21,t2139,t2140,t2147,t2152,t2154,t2155,t2159,t2165,t2174,t2183,t2187,t2193,t2194,t2195,t2199,t22,t2203,t2215,t2219,t2222,t2223,t2239,t2240,t2256,t2257,t2292,t2295,t2297,t23,t2303,t2306,t2307,t2317,t2337,t2338,t2339,t2355,t236,t2361,t2362,t2363,t2367,t237,t2371,t238,t2388,t24,t241,t2414,t2419,t244,t25,t2502,t2519,t2527,t2555,t2556,t2572,t2583,t2598,t26,t2605,t2606,t2612,t2613,t2618,t2619,t262,t264,t2651,t2652,t2671,t2674,t2676,t2683,t2684,t2689,t2694,t2695,t2698,t27,t2701,t2707,t2716,t2719,t2740,t2747,t2754,t28,t2801,t2804,t2813,t2814,t2820,t2831,t2834,t2835,t2838,t2850,t2851,t2953,t2994,t3,t30,t3009,t3022,t3027,t3030,t3036,t3043,t3047,t3057,t3064,t3072,t3080,t3096,t3097,t31,t3109,t3117,t3118,t3121,t3122,t3130,t3131,t3132,t3144,t3147,t3156,t3157,t3170,t32,t3206,t3209,t321,t3210,t3214,t3228,t3229,t3230,t3231,t3232,t3235,t3269,t3270,t3272,t3283,t3290,t3292,t3296,t33,t3305,t3306,t3308,t3313,t3318,t3319,t332,t3327,t3334,t3341,t3349,t335,t3359,t3360,t3376,t3385,t3386,t3395,t3399,t34,t3405,t3409,t3410,t3412,t3417,t3420,t3421,t3423,t3424,t3435,t3437,t3468,t3480,t3481,t3483,t3484,t3493,t3498,t35,t350,t3505,t3524,t3528,t3535,t3544,t3547,t3560,t3563,t3570,t3571,t3576,t3582,t3588,t3590,t3593,t36,t3617,t3620,t3621,t3622,t3628,t3634,t3637,t3638,t3649,t366,t3680,t3681,t3684,t3685,t3689,t3693,t3694,t3708,t3714,t3716,t3723,t3732,t3779,t3782,t3783,t3784,t3790,t3791,t38,t3811,t3817,t3827,t3833,t3834,t3861,t3862,t3863,t3869,t3870,t3871,t3877,t3880,t3882,t3891,t3892,t3898,t39,t3901,t3904,t3910,t3918,t3928,t3934,t3940,t3941,t3942,t3946,t3951,t3957,t3959,t3967,t3972,t3974,t3984,t3985,t3992,t3996,t4,t4007,t4011,t4013,t4015,t4016,t4027,t4062,t4071,t4072,t4076,t4077,t4080,t410,t4108,t4119,t4120,t4134,t4149,t4154,t4160,t4163,t4173,t4175,t4196,t42,t4200,t4219,t4220,t4230,t4231,t4238,t4239,t4242,t4255,t4256,t4257,t4259,t4264,t4266,t4277,t4279,t4280,t4281,t4285,t4287,t4295,t4298,t43,t4304,t4311,t4323,t4324,t4409,t4421,t4437,t4438,t4444,t4447,t4458,t4491,t4496,t4499,t4500,t4504,t4507,t4510,t4513,t4514,t4519,t4520,t4531,t4540,t4541,t4543,t4552,t4554,t4555,t4556,t4560,t4571,t4572,t4576,t4582,t4589,t4595,t46,t4610,t4615,t4620,t4640,t4644,t4650,t4655,t4658,t4663,t4686,t4688,t4699,t47,t4702,t4704,t4705,t4737,t4741,t4744,t4751,t4752,t4758,t4767,t4777,t4780,t4785,t4786,t4789,t4792,t4795,t4814,t4817,t4819,t4822,t4824,t4833,t4848,t4849,t4850,t4851,t4856,t4857,t4860,t4865,t4868,t4869,t4874,t4898,t4911,t4963,t4965,t4974,t4975,t4976,t4977,t4983,t4985,t4986,t4987,t4992,t5,t50,t5005,t5031,t5034,t5035,t5036,t5038,t5039,t5040,t5041,t5042,t5047,t5048,t5049,t5051,t5052,t5056,t5057,t5058,t5069,t5103,t5104,t5105,t5111,t5114,t5117,t5119,t5133,t5134,t5135,t5136,t5139,t5140,t5148,t5150,t5151,t5152,t5155,t5164,t5186,t5189,t5192,t5196,t5204,t5207,t5209,t5210,t5220,t5223,t5224,t5225,t5227,t5230,t5231,t5235,t5240,t5241,t5245,t5246,t5247,t5248,t5252,t5262,t5273,t5276,t5277,t5278,t5281,t5282,t5285,t5286,t5289,t5291,t5314,t5321,t5322,t5330,t5331,t5332,t5335,t5338,t5340,t5345,t5348,t5357,t5365,t5384,t5388,t5400,t5412,t5413,t5426,t5427,t5429,t5433,t5434,t5436,t5437,t5438,t5440,t5441,t5443,t5453,t5460,t5468,t5486,t5488,t5489,t5491,t5504,t5505,t5506,t5507,t5509,t5512,t5515,t5516,t5518,t5520,t5522,t5527,t5528,t5531,t5534,t5538,t5543,t5544,t5550,t5556,t5558,t5561,t5563,t5575,t5578,t5582,t5585,t5588,t5589,t5592,t5594,t5595,t56,t5601,t5612,t5615,t5617,t5619,t5620,t5621,t5626,t5628,t5639,t5654,t5655,t5659,t5662,t5665,t5685,t5687,t5689,t5704,t5705,t5707,t5710,t5711,t5713,t5715,t5722,t5723,t5738,t5739,t5740,t5743,t5751,t5756,t5760,t5762,t5765,t5772,t5773,t5775,t5782,t5785,t5791,t5798,t5799,t5800,t5801,t5809,t5810,t5813,t5822,t5824,t5832,t5833,t5835,t5836,t5845,t5851,t5852,t5853,t5858,t5873,t5876,t5877,t5879,t5884,t5885,t5890,t5892,t5894,t5900,t5919,t5923,t5943,t5944,t5946,t5948,t5951,t5953,t5954,t5958,t5969,t5970,t5975,t5976,t5983,t5985,t5997,t5998,t6,t60,t6001,t6002,t6005,t6007,t6009,t6018,t6020,t6023,t6028,t6030,t6039,t6048,t6054,t6088,t6089,t6101,t6104,t6108,t6110,t6113,t6116,t6117,t6118,t6119,t6122,t6123,t6124,t6147,t6169,t6172,t6179,t6183,t6184,t6185,t6206,t6207,t6210,t6214,t6223,t6226,t6229,t6233,t6234,t6236,t6237,t6240,t6242,t6256,t6289,t6291,t6294,t6300,t6303,t6304,t6317,t6318,t6321,t6323,t6345,t6348,t6356,t6359,t6360,t6361,t6362,t6370,t6379,t6387,t6389,t6391,t6392,t6399,t6401,t6413,t642,t6423,t6425,t643,t6450,t6453,t6459,t6477,t6478,t6485,t649,t6493,t6497,t6508,t6522,t6523,t6529,t6534,t6536,t6538,t6540,t6541,t6561,t6564,t6565,t6587,t6588,t6595,t6598,t6600,t6604,t6606,t6608,t6611,t6613,t6614,t6615,t6616,t6617,t6620,t6623,t6625,t6628,t6631,t6638,t6641,t6647,t6648,t6656,t6657,t6660,t667,t6671,t6674,t6675,t6676,t6677,t6681,t6688,t6689,t6690,t6692,t6694,t6696,t6697,t6698,t6699,t670,t6701,t674,t6753,t6763,t6765,t6767,t6770,t6772,t6774,t6777,t6795,t6801,t6802,t6807,t6809,t6811,t6812,t684,t685,t6851,t6854,t6857,t686,t6860,t6861,t6863,t6864,t6866,t6869,t687,t6871,t6872,t6887,t6892,t6894,t6898,t6899,t6903,t6929,t6930,t6932,t6934,t6936,t6938,t6940,t6942,t6943,t6945,t6949,t6954,t6956,t6961,t6972,t6975,t6976,t6984,t6985,t6986,t6993,t6994,t7,t7004,t7006,t7033,t7047,t7054,t7057,t7058,t7066,t7068,t707,t7070,t7072,t7077,t708,t7086,t7091,t7099,t710,t7100,t7138,t7140,t7142,t7145,t7179,t7181,t7200,t7202,t7204,t721,t7211,t7219,t722,t7223,t7224,t724,t7262,t7266,t7268,t7282,t7288,t7290,t7292,t7293,t7295,t7297,t7298,t7299,t7302,t7304,t7318,t7319,t7322,t7325,t7326,t7331,t7336,t7342,t7349,t7352,t7353,t7354,t7356,t7359,t7362,t7363,t7371,t7372,t7389,t7391,t7395,t7398,t7405,t7416,t7417,t7422,t7424,t7432,t7440,t7443,t7444,t7446,t7448,t7450,t7453,t7466,t7474,t7476,t7478,t7484,t7486,t7487,t7488,t749,t7492,t7494,t7498,t7505,t7521,t7523,t7525,t7527,t7540,t7541,t7545,t7554,t7566,t7568,t7570,t7579,t7581,t7583,t7587,t7598,t7602,t7611,t7613,t7615,t7616,t762,t7621,t7624,t7631,t7632,t7633,t7635,t7637,t7638,t7652,t7655,t7665,t7676,t7678,t768,t7683,t7690,t7693,t7698,t7700,t7702,t7712,t7725,t7727,t7730,t7731,t7733,t7734,t7735,t7740,t7741,t7745,t7746,t7749,t7755,t7757,t777,t7771,t7773,t7776,t7779,t7782,t7784,t7785,t7789,t7790,t7791,t7796,t7797,t7803,t7804,t7805,t7806,t7834,t7835,t7841,t7846,t7851,t7854,t7865,t7868,t7870,t7871,t7872,t7877,t7883,t7888,t7889,t7892,t7894,t7897,t7898,t7900,t7904,t7907,t7910,t7911,t7917,t7919,t792,t7920,t7921,t7922,t7927,t7929,t793,t7931,t7933,t7935,t7936,t7943,t7944,t7945,t7947,t7948,t7952,t7953,t7954,t7955,t7956,t7959,t7968,t7970,t7973,t7974,t7975,t7977,t7978,t7979,t7983,t7984,t7985,t7989,t7990,t7991,t7992,t7993,t7994,t7995,t7996,t7997,t8000,t8001,t8002,t8003,t8004,t8005,t8006,t801,t8012,t8015,t8018,t8019,t802,t8020,t8021,t8022,t8023,t8024,t8025,t8027,t8029,t8031,t8033,t8034,t8035,t8036,t8038,t8040,t8042,t8044,t8045,t8047,t8049,t8051,t808,t813,t819,t821,t850,t855,t874,t878,t941,t948,t951});
end
function tau_c = ft_17(ct)
et398 = ct{1};
et399 = ct{2};
et433 = ct{3};
et434 = ct{4};
et435 = ct{5};
et436 = ct{6};
et439 = ct{7};
et440 = ct{8};
et441 = ct{9};
et442 = ct{10};
et443 = ct{11};
et444 = ct{12};
et445 = ct{13};
et446 = ct{14};
et447 = ct{15};
et448 = ct{16};
t1005 = ct{17};
t1022 = ct{18};
t1196 = ct{19};
t1205 = ct{20};
t1210 = ct{21};
t1212 = ct{22};
t1217 = ct{23};
t1218 = ct{24};
t123 = ct{25};
t1237 = ct{26};
t1238 = ct{27};
t1288 = ct{28};
t1289 = ct{29};
t1302 = ct{30};
t1303 = ct{31};
t1319 = ct{32};
t1320 = ct{33};
t1336 = ct{34};
t1348 = ct{35};
t1350 = ct{36};
t1351 = ct{37};
t1360 = ct{38};
t1369 = ct{39};
t1378 = ct{40};
t1396 = ct{41};
t14 = ct{42};
t140 = ct{43};
t1425 = ct{44};
t1435 = ct{45};
t1456 = ct{46};
t1477 = ct{47};
t1488 = ct{48};
t15 = ct{49};
t1513 = ct{50};
t1539 = ct{51};
t1554 = ct{52};
t1577 = ct{53};
t1578 = ct{54};
t1586 = ct{55};
t1587 = ct{56};
t16 = ct{57};
t1600 = ct{58};
t1606 = ct{59};
t1608 = ct{60};
t1609 = ct{61};
t1629 = ct{62};
t1637 = ct{63};
t1640 = ct{64};
t1641 = ct{65};
t1659 = ct{66};
t1661 = ct{67};
t1666 = ct{68};
t1667 = ct{69};
t1683 = ct{70};
t1686 = ct{71};
t1690 = ct{72};
t1692 = ct{73};
t17 = ct{74};
t1700 = ct{75};
t1701 = ct{76};
t1705 = ct{77};
t1712 = ct{78};
t1758 = ct{79};
t1759 = ct{80};
t1775 = ct{81};
t1776 = ct{82};
t18 = ct{83};
t1861 = ct{84};
t1874 = ct{85};
t1879 = ct{86};
t188 = ct{87};
t1881 = ct{88};
t189 = ct{89};
t1896 = ct{90};
t19 = ct{91};
t1901 = ct{92};
t1941 = ct{93};
t1959 = ct{94};
t1973 = ct{95};
t1993 = ct{96};
t1994 = ct{97};
t2 = ct{98};
t20 = ct{99};
t201 = ct{100};
t202 = ct{101};
t2023 = ct{102};
t2053 = ct{103};
t2060 = ct{104};
t2089 = ct{105};
t2090 = ct{106};
t2098 = ct{107};
t2099 = ct{108};
t21 = ct{109};
t2139 = ct{110};
t2140 = ct{111};
t2147 = ct{112};
t2152 = ct{113};
t2154 = ct{114};
t2155 = ct{115};
t2159 = ct{116};
t2165 = ct{117};
t2174 = ct{118};
t2183 = ct{119};
t2187 = ct{120};
t2193 = ct{121};
t2194 = ct{122};
t2195 = ct{123};
t2199 = ct{124};
t22 = ct{125};
t2203 = ct{126};
t2215 = ct{127};
t2219 = ct{128};
t2222 = ct{129};
t2223 = ct{130};
t2239 = ct{131};
t2240 = ct{132};
t2256 = ct{133};
t2257 = ct{134};
t2292 = ct{135};
t2295 = ct{136};
t2297 = ct{137};
t23 = ct{138};
t2303 = ct{139};
t2306 = ct{140};
t2307 = ct{141};
t2317 = ct{142};
t2337 = ct{143};
t2338 = ct{144};
t2339 = ct{145};
t2355 = ct{146};
t236 = ct{147};
t2361 = ct{148};
t2362 = ct{149};
t2363 = ct{150};
t2367 = ct{151};
t237 = ct{152};
t2371 = ct{153};
t238 = ct{154};
t2388 = ct{155};
t24 = ct{156};
t241 = ct{157};
t2414 = ct{158};
t2419 = ct{159};
t244 = ct{160};
t25 = ct{161};
t2502 = ct{162};
t2519 = ct{163};
t2527 = ct{164};
t2555 = ct{165};
t2556 = ct{166};
t2572 = ct{167};
t2583 = ct{168};
t2598 = ct{169};
t26 = ct{170};
t2605 = ct{171};
t2606 = ct{172};
t2612 = ct{173};
t2613 = ct{174};
t2618 = ct{175};
t2619 = ct{176};
t262 = ct{177};
t264 = ct{178};
t2651 = ct{179};
t2652 = ct{180};
t2671 = ct{181};
t2674 = ct{182};
t2676 = ct{183};
t2683 = ct{184};
t2684 = ct{185};
t2689 = ct{186};
t2694 = ct{187};
t2695 = ct{188};
t2698 = ct{189};
t27 = ct{190};
t2701 = ct{191};
t2707 = ct{192};
t2716 = ct{193};
t2719 = ct{194};
t2740 = ct{195};
t2747 = ct{196};
t2754 = ct{197};
t28 = ct{198};
t2801 = ct{199};
t2804 = ct{200};
t2813 = ct{201};
t2814 = ct{202};
t2820 = ct{203};
t2831 = ct{204};
t2834 = ct{205};
t2835 = ct{206};
t2838 = ct{207};
t2850 = ct{208};
t2851 = ct{209};
t2953 = ct{210};
t2994 = ct{211};
t3 = ct{212};
t30 = ct{213};
t3009 = ct{214};
t3022 = ct{215};
t3027 = ct{216};
t3030 = ct{217};
t3036 = ct{218};
t3043 = ct{219};
t3047 = ct{220};
t3057 = ct{221};
t3064 = ct{222};
t3072 = ct{223};
t3080 = ct{224};
t3096 = ct{225};
t3097 = ct{226};
t31 = ct{227};
t3109 = ct{228};
t3117 = ct{229};
t3118 = ct{230};
t3121 = ct{231};
t3122 = ct{232};
t3130 = ct{233};
t3131 = ct{234};
t3132 = ct{235};
t3144 = ct{236};
t3147 = ct{237};
t3156 = ct{238};
t3157 = ct{239};
t3170 = ct{240};
t32 = ct{241};
t3206 = ct{242};
t3209 = ct{243};
t321 = ct{244};
t3210 = ct{245};
t3214 = ct{246};
t3228 = ct{247};
t3229 = ct{248};
t3230 = ct{249};
t3231 = ct{250};
t3232 = ct{251};
t3235 = ct{252};
t3269 = ct{253};
t3270 = ct{254};
t3272 = ct{255};
t3283 = ct{256};
t3290 = ct{257};
t3292 = ct{258};
t3296 = ct{259};
t33 = ct{260};
t3305 = ct{261};
t3306 = ct{262};
t3308 = ct{263};
t3313 = ct{264};
t3318 = ct{265};
t3319 = ct{266};
t332 = ct{267};
t3327 = ct{268};
t3334 = ct{269};
t3341 = ct{270};
t3349 = ct{271};
t335 = ct{272};
t3359 = ct{273};
t3360 = ct{274};
t3376 = ct{275};
t3385 = ct{276};
t3386 = ct{277};
t3395 = ct{278};
t3399 = ct{279};
t34 = ct{280};
t3405 = ct{281};
t3409 = ct{282};
t3410 = ct{283};
t3412 = ct{284};
t3417 = ct{285};
t3420 = ct{286};
t3421 = ct{287};
t3423 = ct{288};
t3424 = ct{289};
t3435 = ct{290};
t3437 = ct{291};
t3468 = ct{292};
t3480 = ct{293};
t3481 = ct{294};
t3483 = ct{295};
t3484 = ct{296};
t3493 = ct{297};
t3498 = ct{298};
t35 = ct{299};
t350 = ct{300};
t3505 = ct{301};
t3524 = ct{302};
t3528 = ct{303};
t3535 = ct{304};
t3544 = ct{305};
t3547 = ct{306};
t3560 = ct{307};
t3563 = ct{308};
t3570 = ct{309};
t3571 = ct{310};
t3576 = ct{311};
t3582 = ct{312};
t3588 = ct{313};
t3590 = ct{314};
t3593 = ct{315};
t36 = ct{316};
t3617 = ct{317};
t3620 = ct{318};
t3621 = ct{319};
t3622 = ct{320};
t3628 = ct{321};
t3634 = ct{322};
t3637 = ct{323};
t3638 = ct{324};
t3649 = ct{325};
t366 = ct{326};
t3680 = ct{327};
t3681 = ct{328};
t3684 = ct{329};
t3685 = ct{330};
t3689 = ct{331};
t3693 = ct{332};
t3694 = ct{333};
t3708 = ct{334};
t3714 = ct{335};
t3716 = ct{336};
t3723 = ct{337};
t3732 = ct{338};
t3779 = ct{339};
t3782 = ct{340};
t3783 = ct{341};
t3784 = ct{342};
t3790 = ct{343};
t3791 = ct{344};
t38 = ct{345};
t3811 = ct{346};
t3817 = ct{347};
t3827 = ct{348};
t3833 = ct{349};
t3834 = ct{350};
t3861 = ct{351};
t3862 = ct{352};
t3863 = ct{353};
t3869 = ct{354};
t3870 = ct{355};
t3871 = ct{356};
t3877 = ct{357};
t3880 = ct{358};
t3882 = ct{359};
t3891 = ct{360};
t3892 = ct{361};
t3898 = ct{362};
t39 = ct{363};
t3901 = ct{364};
t3904 = ct{365};
t3910 = ct{366};
t3918 = ct{367};
t3928 = ct{368};
t3934 = ct{369};
t3940 = ct{370};
t3941 = ct{371};
t3942 = ct{372};
t3946 = ct{373};
t3951 = ct{374};
t3957 = ct{375};
t3959 = ct{376};
t3967 = ct{377};
t3972 = ct{378};
t3974 = ct{379};
t3984 = ct{380};
t3985 = ct{381};
t3992 = ct{382};
t3996 = ct{383};
t4 = ct{384};
t4007 = ct{385};
t4011 = ct{386};
t4013 = ct{387};
t4015 = ct{388};
t4016 = ct{389};
t4027 = ct{390};
t4062 = ct{391};
t4071 = ct{392};
t4072 = ct{393};
t4076 = ct{394};
t4077 = ct{395};
t4080 = ct{396};
t410 = ct{397};
t4108 = ct{398};
t4119 = ct{399};
t4120 = ct{400};
t4134 = ct{401};
t4149 = ct{402};
t4154 = ct{403};
t4160 = ct{404};
t4163 = ct{405};
t4173 = ct{406};
t4175 = ct{407};
t4196 = ct{408};
t42 = ct{409};
t4200 = ct{410};
t4219 = ct{411};
t4220 = ct{412};
t4230 = ct{413};
t4231 = ct{414};
t4238 = ct{415};
t4239 = ct{416};
t4242 = ct{417};
t4255 = ct{418};
t4256 = ct{419};
t4257 = ct{420};
t4259 = ct{421};
t4264 = ct{422};
t4266 = ct{423};
t4277 = ct{424};
t4279 = ct{425};
t4280 = ct{426};
t4281 = ct{427};
t4285 = ct{428};
t4287 = ct{429};
t4295 = ct{430};
t4298 = ct{431};
t43 = ct{432};
t4304 = ct{433};
t4311 = ct{434};
t4323 = ct{435};
t4324 = ct{436};
t4409 = ct{437};
t4421 = ct{438};
t4437 = ct{439};
t4438 = ct{440};
t4444 = ct{441};
t4447 = ct{442};
t4458 = ct{443};
t4491 = ct{444};
t4496 = ct{445};
t4499 = ct{446};
t4500 = ct{447};
t4504 = ct{448};
t4507 = ct{449};
t4510 = ct{450};
t4513 = ct{451};
t4514 = ct{452};
t4519 = ct{453};
t4520 = ct{454};
t4531 = ct{455};
t4540 = ct{456};
t4541 = ct{457};
t4543 = ct{458};
t4552 = ct{459};
t4554 = ct{460};
t4555 = ct{461};
t4556 = ct{462};
t4560 = ct{463};
t4571 = ct{464};
t4572 = ct{465};
t4576 = ct{466};
t4582 = ct{467};
t4589 = ct{468};
t4595 = ct{469};
t46 = ct{470};
t4610 = ct{471};
t4615 = ct{472};
t4620 = ct{473};
t4640 = ct{474};
t4644 = ct{475};
t4650 = ct{476};
t4655 = ct{477};
t4658 = ct{478};
t4663 = ct{479};
t4686 = ct{480};
t4688 = ct{481};
t4699 = ct{482};
t47 = ct{483};
t4702 = ct{484};
t4704 = ct{485};
t4705 = ct{486};
t4737 = ct{487};
t4741 = ct{488};
t4744 = ct{489};
t4751 = ct{490};
t4752 = ct{491};
t4758 = ct{492};
t4767 = ct{493};
t4777 = ct{494};
t4780 = ct{495};
t4785 = ct{496};
t4786 = ct{497};
t4789 = ct{498};
t4792 = ct{499};
t4795 = ct{500};
t4814 = ct{501};
t4817 = ct{502};
t4819 = ct{503};
t4822 = ct{504};
t4824 = ct{505};
t4833 = ct{506};
t4848 = ct{507};
t4849 = ct{508};
t4850 = ct{509};
t4851 = ct{510};
t4856 = ct{511};
t4857 = ct{512};
t4860 = ct{513};
t4865 = ct{514};
t4868 = ct{515};
t4869 = ct{516};
t4874 = ct{517};
t4898 = ct{518};
t4911 = ct{519};
t4963 = ct{520};
t4965 = ct{521};
t4974 = ct{522};
t4975 = ct{523};
t4976 = ct{524};
t4977 = ct{525};
t4983 = ct{526};
t4985 = ct{527};
t4986 = ct{528};
t4987 = ct{529};
t4992 = ct{530};
t5 = ct{531};
t50 = ct{532};
t5005 = ct{533};
t5031 = ct{534};
t5034 = ct{535};
t5035 = ct{536};
t5036 = ct{537};
t5038 = ct{538};
t5039 = ct{539};
t5040 = ct{540};
t5041 = ct{541};
t5042 = ct{542};
t5047 = ct{543};
t5048 = ct{544};
t5049 = ct{545};
t5051 = ct{546};
t5052 = ct{547};
t5056 = ct{548};
t5057 = ct{549};
t5058 = ct{550};
t5069 = ct{551};
t5103 = ct{552};
t5104 = ct{553};
t5105 = ct{554};
t5111 = ct{555};
t5114 = ct{556};
t5117 = ct{557};
t5119 = ct{558};
t5133 = ct{559};
t5134 = ct{560};
t5135 = ct{561};
t5136 = ct{562};
t5139 = ct{563};
t5140 = ct{564};
t5148 = ct{565};
t5150 = ct{566};
t5151 = ct{567};
t5152 = ct{568};
t5155 = ct{569};
t5164 = ct{570};
t5186 = ct{571};
t5189 = ct{572};
t5192 = ct{573};
t5196 = ct{574};
t5204 = ct{575};
t5207 = ct{576};
t5209 = ct{577};
t5210 = ct{578};
t5220 = ct{579};
t5223 = ct{580};
t5224 = ct{581};
t5225 = ct{582};
t5227 = ct{583};
t5230 = ct{584};
t5231 = ct{585};
t5235 = ct{586};
t5240 = ct{587};
t5241 = ct{588};
t5245 = ct{589};
t5246 = ct{590};
t5247 = ct{591};
t5248 = ct{592};
t5252 = ct{593};
t5262 = ct{594};
t5273 = ct{595};
t5276 = ct{596};
t5277 = ct{597};
t5278 = ct{598};
t5281 = ct{599};
t5282 = ct{600};
t5285 = ct{601};
t5286 = ct{602};
t5289 = ct{603};
t5291 = ct{604};
t5314 = ct{605};
t5321 = ct{606};
t5322 = ct{607};
t5330 = ct{608};
t5331 = ct{609};
t5332 = ct{610};
t5335 = ct{611};
t5338 = ct{612};
t5340 = ct{613};
t5345 = ct{614};
t5348 = ct{615};
t5357 = ct{616};
t5365 = ct{617};
t5384 = ct{618};
t5388 = ct{619};
t5400 = ct{620};
t5412 = ct{621};
t5413 = ct{622};
t5426 = ct{623};
t5427 = ct{624};
t5429 = ct{625};
t5433 = ct{626};
t5434 = ct{627};
t5436 = ct{628};
t5437 = ct{629};
t5438 = ct{630};
t5440 = ct{631};
t5441 = ct{632};
t5443 = ct{633};
t5453 = ct{634};
t5460 = ct{635};
t5468 = ct{636};
t5486 = ct{637};
t5488 = ct{638};
t5489 = ct{639};
t5491 = ct{640};
t5504 = ct{641};
t5505 = ct{642};
t5506 = ct{643};
t5507 = ct{644};
t5509 = ct{645};
t5512 = ct{646};
t5515 = ct{647};
t5516 = ct{648};
t5518 = ct{649};
t5520 = ct{650};
t5522 = ct{651};
t5527 = ct{652};
t5528 = ct{653};
t5531 = ct{654};
t5534 = ct{655};
t5538 = ct{656};
t5543 = ct{657};
t5544 = ct{658};
t5550 = ct{659};
t5556 = ct{660};
t5558 = ct{661};
t5561 = ct{662};
t5563 = ct{663};
t5575 = ct{664};
t5578 = ct{665};
t5582 = ct{666};
t5585 = ct{667};
t5588 = ct{668};
t5589 = ct{669};
t5592 = ct{670};
t5594 = ct{671};
t5595 = ct{672};
t56 = ct{673};
t5601 = ct{674};
t5612 = ct{675};
t5615 = ct{676};
t5617 = ct{677};
t5619 = ct{678};
t5620 = ct{679};
t5621 = ct{680};
t5626 = ct{681};
t5628 = ct{682};
t5639 = ct{683};
t5654 = ct{684};
t5655 = ct{685};
t5659 = ct{686};
t5662 = ct{687};
t5665 = ct{688};
t5685 = ct{689};
t5687 = ct{690};
t5689 = ct{691};
t5704 = ct{692};
t5705 = ct{693};
t5707 = ct{694};
t5710 = ct{695};
t5711 = ct{696};
t5713 = ct{697};
t5715 = ct{698};
t5722 = ct{699};
t5723 = ct{700};
t5738 = ct{701};
t5739 = ct{702};
t5740 = ct{703};
t5743 = ct{704};
t5751 = ct{705};
t5756 = ct{706};
t5760 = ct{707};
t5762 = ct{708};
t5765 = ct{709};
t5772 = ct{710};
t5773 = ct{711};
t5775 = ct{712};
t5782 = ct{713};
t5785 = ct{714};
t5791 = ct{715};
t5798 = ct{716};
t5799 = ct{717};
t5800 = ct{718};
t5801 = ct{719};
t5809 = ct{720};
t5810 = ct{721};
t5813 = ct{722};
t5822 = ct{723};
t5824 = ct{724};
t5832 = ct{725};
t5833 = ct{726};
t5835 = ct{727};
t5836 = ct{728};
t5845 = ct{729};
t5851 = ct{730};
t5852 = ct{731};
t5853 = ct{732};
t5858 = ct{733};
t5873 = ct{734};
t5876 = ct{735};
t5877 = ct{736};
t5879 = ct{737};
t5884 = ct{738};
t5885 = ct{739};
t5890 = ct{740};
t5892 = ct{741};
t5894 = ct{742};
t5900 = ct{743};
t5919 = ct{744};
t5923 = ct{745};
t5943 = ct{746};
t5944 = ct{747};
t5946 = ct{748};
t5948 = ct{749};
t5951 = ct{750};
t5953 = ct{751};
t5954 = ct{752};
t5958 = ct{753};
t5969 = ct{754};
t5970 = ct{755};
t5975 = ct{756};
t5976 = ct{757};
t5983 = ct{758};
t5985 = ct{759};
t5997 = ct{760};
t5998 = ct{761};
t6 = ct{762};
t60 = ct{763};
t6001 = ct{764};
t6002 = ct{765};
t6005 = ct{766};
t6007 = ct{767};
t6009 = ct{768};
t6018 = ct{769};
t6020 = ct{770};
t6023 = ct{771};
t6028 = ct{772};
t6030 = ct{773};
t6039 = ct{774};
t6048 = ct{775};
t6054 = ct{776};
t6088 = ct{777};
t6089 = ct{778};
t6101 = ct{779};
t6104 = ct{780};
t6108 = ct{781};
t6110 = ct{782};
t6113 = ct{783};
t6116 = ct{784};
t6117 = ct{785};
t6118 = ct{786};
t6119 = ct{787};
t6122 = ct{788};
t6123 = ct{789};
t6124 = ct{790};
t6147 = ct{791};
t6169 = ct{792};
t6172 = ct{793};
t6179 = ct{794};
t6183 = ct{795};
t6184 = ct{796};
t6185 = ct{797};
t6206 = ct{798};
t6207 = ct{799};
t6210 = ct{800};
t6214 = ct{801};
t6223 = ct{802};
t6226 = ct{803};
t6229 = ct{804};
t6233 = ct{805};
t6234 = ct{806};
t6236 = ct{807};
t6237 = ct{808};
t6240 = ct{809};
t6242 = ct{810};
t6256 = ct{811};
t6289 = ct{812};
t6291 = ct{813};
t6294 = ct{814};
t6300 = ct{815};
t6303 = ct{816};
t6304 = ct{817};
t6317 = ct{818};
t6318 = ct{819};
t6321 = ct{820};
t6323 = ct{821};
t6345 = ct{822};
t6348 = ct{823};
t6356 = ct{824};
t6359 = ct{825};
t6360 = ct{826};
t6361 = ct{827};
t6362 = ct{828};
t6370 = ct{829};
t6379 = ct{830};
t6387 = ct{831};
t6389 = ct{832};
t6391 = ct{833};
t6392 = ct{834};
t6399 = ct{835};
t6401 = ct{836};
t6413 = ct{837};
t642 = ct{838};
t6423 = ct{839};
t6425 = ct{840};
t643 = ct{841};
t6450 = ct{842};
t6453 = ct{843};
t6459 = ct{844};
t6477 = ct{845};
t6478 = ct{846};
t6485 = ct{847};
t649 = ct{848};
t6493 = ct{849};
t6497 = ct{850};
t6508 = ct{851};
t6522 = ct{852};
t6523 = ct{853};
t6529 = ct{854};
t6534 = ct{855};
t6536 = ct{856};
t6538 = ct{857};
t6540 = ct{858};
t6541 = ct{859};
t6561 = ct{860};
t6564 = ct{861};
t6565 = ct{862};
t6587 = ct{863};
t6588 = ct{864};
t6595 = ct{865};
t6598 = ct{866};
t6600 = ct{867};
t6604 = ct{868};
t6606 = ct{869};
t6608 = ct{870};
t6611 = ct{871};
t6613 = ct{872};
t6614 = ct{873};
t6615 = ct{874};
t6616 = ct{875};
t6617 = ct{876};
t6620 = ct{877};
t6623 = ct{878};
t6625 = ct{879};
t6628 = ct{880};
t6631 = ct{881};
t6638 = ct{882};
t6641 = ct{883};
t6647 = ct{884};
t6648 = ct{885};
t6656 = ct{886};
t6657 = ct{887};
t6660 = ct{888};
t667 = ct{889};
t6671 = ct{890};
t6674 = ct{891};
t6675 = ct{892};
t6676 = ct{893};
t6677 = ct{894};
t6681 = ct{895};
t6688 = ct{896};
t6689 = ct{897};
t6690 = ct{898};
t6692 = ct{899};
t6694 = ct{900};
t6696 = ct{901};
t6697 = ct{902};
t6698 = ct{903};
t6699 = ct{904};
t670 = ct{905};
t6701 = ct{906};
t674 = ct{907};
t6753 = ct{908};
t6763 = ct{909};
t6765 = ct{910};
t6767 = ct{911};
t6770 = ct{912};
t6772 = ct{913};
t6774 = ct{914};
t6777 = ct{915};
t6795 = ct{916};
t6801 = ct{917};
t6802 = ct{918};
t6807 = ct{919};
t6809 = ct{920};
t6811 = ct{921};
t6812 = ct{922};
t684 = ct{923};
t685 = ct{924};
t6851 = ct{925};
t6854 = ct{926};
t6857 = ct{927};
t686 = ct{928};
t6860 = ct{929};
t6861 = ct{930};
t6863 = ct{931};
t6864 = ct{932};
t6866 = ct{933};
t6869 = ct{934};
t687 = ct{935};
t6871 = ct{936};
t6872 = ct{937};
t6887 = ct{938};
t6892 = ct{939};
t6894 = ct{940};
t6898 = ct{941};
t6899 = ct{942};
t6903 = ct{943};
t6929 = ct{944};
t6930 = ct{945};
t6932 = ct{946};
t6934 = ct{947};
t6936 = ct{948};
t6938 = ct{949};
t6940 = ct{950};
t6942 = ct{951};
t6943 = ct{952};
t6945 = ct{953};
t6949 = ct{954};
t6954 = ct{955};
t6956 = ct{956};
t6961 = ct{957};
t6972 = ct{958};
t6975 = ct{959};
t6976 = ct{960};
t6984 = ct{961};
t6985 = ct{962};
t6986 = ct{963};
t6993 = ct{964};
t6994 = ct{965};
t7 = ct{966};
t7004 = ct{967};
t7006 = ct{968};
t7033 = ct{969};
t7047 = ct{970};
t7054 = ct{971};
t7057 = ct{972};
t7058 = ct{973};
t7066 = ct{974};
t7068 = ct{975};
t707 = ct{976};
t7070 = ct{977};
t7072 = ct{978};
t7077 = ct{979};
t708 = ct{980};
t7086 = ct{981};
t7091 = ct{982};
t7099 = ct{983};
t710 = ct{984};
t7100 = ct{985};
t7138 = ct{986};
t7140 = ct{987};
t7142 = ct{988};
t7145 = ct{989};
t7179 = ct{990};
t7181 = ct{991};
t7200 = ct{992};
t7202 = ct{993};
t7204 = ct{994};
t721 = ct{995};
t7211 = ct{996};
t7219 = ct{997};
t722 = ct{998};
t7223 = ct{999};
t7224 = ct{1000};
t724 = ct{1001};
t7262 = ct{1002};
t7266 = ct{1003};
t7268 = ct{1004};
t7282 = ct{1005};
t7288 = ct{1006};
t7290 = ct{1007};
t7292 = ct{1008};
t7293 = ct{1009};
t7295 = ct{1010};
t7297 = ct{1011};
t7298 = ct{1012};
t7299 = ct{1013};
t7302 = ct{1014};
t7304 = ct{1015};
t7318 = ct{1016};
t7319 = ct{1017};
t7322 = ct{1018};
t7325 = ct{1019};
t7326 = ct{1020};
t7331 = ct{1021};
t7336 = ct{1022};
t7342 = ct{1023};
t7349 = ct{1024};
t7352 = ct{1025};
t7353 = ct{1026};
t7354 = ct{1027};
t7356 = ct{1028};
t7359 = ct{1029};
t7362 = ct{1030};
t7363 = ct{1031};
t7371 = ct{1032};
t7372 = ct{1033};
t7389 = ct{1034};
t7391 = ct{1035};
t7395 = ct{1036};
t7398 = ct{1037};
t7405 = ct{1038};
t7416 = ct{1039};
t7417 = ct{1040};
t7422 = ct{1041};
t7424 = ct{1042};
t7432 = ct{1043};
t7440 = ct{1044};
t7443 = ct{1045};
t7444 = ct{1046};
t7446 = ct{1047};
t7448 = ct{1048};
t7450 = ct{1049};
t7453 = ct{1050};
t7466 = ct{1051};
t7474 = ct{1052};
t7476 = ct{1053};
t7478 = ct{1054};
t7484 = ct{1055};
t7486 = ct{1056};
t7487 = ct{1057};
t7488 = ct{1058};
t749 = ct{1059};
t7492 = ct{1060};
t7494 = ct{1061};
t7498 = ct{1062};
t7505 = ct{1063};
t7521 = ct{1064};
t7523 = ct{1065};
t7525 = ct{1066};
t7527 = ct{1067};
t7540 = ct{1068};
t7541 = ct{1069};
t7545 = ct{1070};
t7554 = ct{1071};
t7566 = ct{1072};
t7568 = ct{1073};
t7570 = ct{1074};
t7579 = ct{1075};
t7581 = ct{1076};
t7583 = ct{1077};
t7587 = ct{1078};
t7598 = ct{1079};
t7602 = ct{1080};
t7611 = ct{1081};
t7613 = ct{1082};
t7615 = ct{1083};
t7616 = ct{1084};
t762 = ct{1085};
t7621 = ct{1086};
t7624 = ct{1087};
t7631 = ct{1088};
t7632 = ct{1089};
t7633 = ct{1090};
t7635 = ct{1091};
t7637 = ct{1092};
t7638 = ct{1093};
t7652 = ct{1094};
t7655 = ct{1095};
t7665 = ct{1096};
t7676 = ct{1097};
t7678 = ct{1098};
t768 = ct{1099};
t7683 = ct{1100};
t7690 = ct{1101};
t7693 = ct{1102};
t7698 = ct{1103};
t7700 = ct{1104};
t7702 = ct{1105};
t7712 = ct{1106};
t7725 = ct{1107};
t7727 = ct{1108};
t7730 = ct{1109};
t7731 = ct{1110};
t7733 = ct{1111};
t7734 = ct{1112};
t7735 = ct{1113};
t7740 = ct{1114};
t7741 = ct{1115};
t7745 = ct{1116};
t7746 = ct{1117};
t7749 = ct{1118};
t7755 = ct{1119};
t7757 = ct{1120};
t777 = ct{1121};
t7771 = ct{1122};
t7773 = ct{1123};
t7776 = ct{1124};
t7779 = ct{1125};
t7782 = ct{1126};
t7784 = ct{1127};
t7785 = ct{1128};
t7789 = ct{1129};
t7790 = ct{1130};
t7791 = ct{1131};
t7796 = ct{1132};
t7797 = ct{1133};
t7803 = ct{1134};
t7804 = ct{1135};
t7805 = ct{1136};
t7806 = ct{1137};
t7834 = ct{1138};
t7835 = ct{1139};
t7841 = ct{1140};
t7846 = ct{1141};
t7851 = ct{1142};
t7854 = ct{1143};
t7865 = ct{1144};
t7868 = ct{1145};
t7870 = ct{1146};
t7871 = ct{1147};
t7872 = ct{1148};
t7877 = ct{1149};
t7883 = ct{1150};
t7888 = ct{1151};
t7889 = ct{1152};
t7892 = ct{1153};
t7894 = ct{1154};
t7897 = ct{1155};
t7898 = ct{1156};
t7900 = ct{1157};
t7904 = ct{1158};
t7907 = ct{1159};
t7910 = ct{1160};
t7911 = ct{1161};
t7917 = ct{1162};
t7919 = ct{1163};
t792 = ct{1164};
t7920 = ct{1165};
t7921 = ct{1166};
t7922 = ct{1167};
t7927 = ct{1168};
t7929 = ct{1169};
t793 = ct{1170};
t7931 = ct{1171};
t7933 = ct{1172};
t7935 = ct{1173};
t7936 = ct{1174};
t7943 = ct{1175};
t7944 = ct{1176};
t7945 = ct{1177};
t7947 = ct{1178};
t7948 = ct{1179};
t7952 = ct{1180};
t7953 = ct{1181};
t7954 = ct{1182};
t7955 = ct{1183};
t7956 = ct{1184};
t7959 = ct{1185};
t7968 = ct{1186};
t7970 = ct{1187};
t7973 = ct{1188};
t7974 = ct{1189};
t7975 = ct{1190};
t7977 = ct{1191};
t7978 = ct{1192};
t7979 = ct{1193};
t7983 = ct{1194};
t7984 = ct{1195};
t7985 = ct{1196};
t7989 = ct{1197};
t7990 = ct{1198};
t7991 = ct{1199};
t7992 = ct{1200};
t7993 = ct{1201};
t7994 = ct{1202};
t7995 = ct{1203};
t7996 = ct{1204};
t7997 = ct{1205};
t8000 = ct{1206};
t8001 = ct{1207};
t8002 = ct{1208};
t8003 = ct{1209};
t8004 = ct{1210};
t8005 = ct{1211};
t8006 = ct{1212};
t801 = ct{1213};
t8012 = ct{1214};
t8015 = ct{1215};
t8018 = ct{1216};
t8019 = ct{1217};
t802 = ct{1218};
t8020 = ct{1219};
t8021 = ct{1220};
t8022 = ct{1221};
t8023 = ct{1222};
t8024 = ct{1223};
t8025 = ct{1224};
t8027 = ct{1225};
t8029 = ct{1226};
t8031 = ct{1227};
t8033 = ct{1228};
t8034 = ct{1229};
t8035 = ct{1230};
t8036 = ct{1231};
t8038 = ct{1232};
t8040 = ct{1233};
t8042 = ct{1234};
t8044 = ct{1235};
t8045 = ct{1236};
t8047 = ct{1237};
t8049 = ct{1238};
t8051 = ct{1239};
t808 = ct{1240};
t813 = ct{1241};
t819 = ct{1242};
t821 = ct{1243};
t850 = ct{1244};
t855 = ct{1245};
t874 = ct{1246};
t878 = ct{1247};
t941 = ct{1248};
t948 = ct{1249};
t951 = ct{1250};
et449 = t16.*t19.*t20.*t50.*t189.*(-3.279367663374749e-19)-t14.*t15.*t17.*t21.*t50.*t189.*7.075931802640439e-19;
et450 = t14.*t17.*t20.*t21.*t50.*t189.*(-1.190170786299927e-18)-t15.*t17.*t19.*t21.*t50.*t189.*1.190170786299927e-18;
et451 = t19.*t20.*t21.*t22.*t50.*t189.*(-3.226512155691387e-19);
et452 = -t4615+t4640-t5252+t5427-t5791+t6089+t6851+t7652+t7655+t7683+t7755+t3209.*(-t5772-t5773+t6522+t6523+t28.*t6620.*(t3235-t3535)+t34.*t6617.*(t3235-t3535))+t4175.*t5224.*(t2694-t2701+t3036-t3043).*1.08769e-2+t3784.*t5951.*(t2694-t2701+t3036-t3043).*1.08769e-2;
et453 = t3918.*t6561.*(t2694-t2701+t3036-t3043).*7.26735e-3+t3784.*t3901.*(et448+et449+et450+et451).*1.08769e-2+t3901.*t5713.*(t1513+t1879+t2598+t2820+t2834+t3117+t3118).*7.26735e-3+t50.*t189.*(t5563+t6360+t6361+t6362+t6795).*9.543032792050485e-17;
et454 = t4.*t8012+(t2.*t8023)./2.0+(t3.*t8024)./2.0-t6.*t8029+(t6.*t8051)./2.0+(t5.*(et439+et440+et441))./2.0-t2.*(et442+et443)-t3.*(et444+et445);
et455 = t4.*(t5388+t5491-t6984-t6985-t7099-t7100+t7432+t7478+t7488+t7927+t7929-t7943+t4822.*(t6767+t6001.*(t1896-t3232)+t3985.*(t3424-t3437+t4552+t4556+t3942.*(t1896-t3232).*5.7e-7+t3946.*(t1896-t3232).*4.0e-8))+t7933.*(t2674-t2676+t3022-t3027)+t7417.*(et446+et447)+t3877.*t7398.*(t1488+t1874+t2519+t2740+t2747+t3096+t3097)).*(-1.0./2.0)+t5.*(et452+et453);
et456 = -t7.*(t7474+t7476+t7771-t7773+t7352.*(t1456-t2355)+t3047.*(t6389-t6391-t6675-t6676+t3057.*(t4752+t3942.*(t2694-t2701+t3036-t3043).*1.02e-6)+t5520.*(t1477-t2502)))+(t7.*(t7486+t7487+t7907+t7947+t7948-t2994.*(-t6677+t6681+t3057.*(-t3423+t4543+t3946.*(t1896-t3232).*1.02e-6))))./2.0;
et457 = t6345+t7292+t4824.*(t4737+t4744+t4751+t3942.*(t2694-t2701+t3036-t3043).*5.7e-7)+t3996.*(t5231+t5235-t5273+t5278+t5282-t5285+t4777.*(t2694-t2701+t3036-t3043).*5.7e-7+t4780.*(t2694-t2701+t3036-t3043).*4.0e-8);
et458 = t3992.*(-t5152+t5230+t5241+t5276-t5277-t5281+t5286+(t4865.*(t1861-t3214))./1.0e+8+(t3901.*(t951+t16.*(-t1881+t3121+t3269)))./1.0e+8+(t4080.*(t2694-t2701+t3036-t3043))./1.0e+8+t4777.*(t2694-t2701+t3036-t3043).*4.0e-8+t4780.*(t2694-t2701+t3036-t3043).*2.4e-7);
et459 = t4814.*(-t4437-t4438+t4741+t4767+t3942.*(t2694-t2701+t3036-t3043).*4.0e-8+t3946.*(t2694-t2701+t3036-t3043).*2.4e-7);
et460 = t3483.*(et457+et458+et459)-t4080.*(t6887+t3985.*(t4737+t4744+t4751+t3942.*(t2694-t2701+t3036-t3043).*5.7e-7)+t6088.*(t1896-t3232))+t2338.*t7352+t2297.*t7931-t2297.*t7952+t3483.*t7954-t4080.*t7440;
et461 = (t1861-t3214).*(t6993+t7293+t7349+t7566-t6088.*(t1005+t26.*(t1941-t3308+t39.*t1022.*(t855-t878).*2.196325630278387e-1))-t4817.*(t4737+t4744+t4751+t3942.*(t2694-t2701+t3036-t3043).*5.7e-7));
et462 = t2338.*(-t6123+t6359+t3057.*(-t4437-t4438+t4741+t4767+t3942.*(t2694-t2701+t3036-t3043).*4.0e-8+t3946.*(t2694-t2701+t3036-t3043).*2.4e-7))-t7953.*(t1861-t3214)-t7443.*(t951+t16.*(-t1881+t3121+t3269));
et463 = -(t951+t16.*(-t1881+t3121+t3269)).*(t6214+t3996.*(t4737+t4744+t4751+t3942.*(t2694-t2701+t3036-t3043).*5.7e-7)+t3992.*(-t4437-t4438+t4741+t4767+t3942.*(t2694-t2701+t3036-t3043).*4.0e-8+t3946.*(t2694-t2701+t3036-t3043).*2.4e-7));
et464 = t4304.*(t4758.*(t1861-t3214)+t2297.*(t642+t643-t667+t674+t1587+t1606+t1608+t1609+t2295+t2671+t2683+t2684-t2695+t3272+t3290-t3296+t3576+t3582+t3588-t3593+t4015+t4016)).*(t2694-t2701+t3036-t3043).*7.26735e-3+t7371.*(t2694-t2701+t3036-t3043).*(t1513+t1879+t2598+t2820+t2834+t3117+t3118).*7.26735e-3+t3901.*t4304.*t6631.*7.26735e-3;
et465 = t3901.*t7372.*(t1513+t1879+t2598+t2820+t2834+t3117+t3118).*7.26735e-3-t4860.*t6631.*(t1513+t1879+t2598+t2820+t2834+t3117+t3118).*7.26735e-3+t4865.*(t4758.*(t1861-t3214)+t2297.*(t642+t643-t667+t674+t1587+t1606+t1608+t1609+t2295+t2671+t2683+t2684-t2695+t3272+t3290-t3296+t3576+t3582+t3588-t3593+t4015+t4016)).*(t1513+t1879+t2598+t2820+t2834+t3117+t3118).*7.26735e-3;
et466 = t236.*t241.*t4421.*t4655.*(-4.788365138921021e-91);
et467 = t236.*t241.*t4589.*t4705.*4.788365138921021e-91;
et468 = t4688-t5036+t5042-t5164+t4865.*(t1861-t3214).*7.83e-6+t3901.*(t951+t16.*(-t1881+t3121+t3269)).*7.83e-6+t4080.*(t2694-t2701+t3036-t3043).*7.83e-6;
et469 = t3901.*(-t1901+t3122+t3270).*3.24e-6;
et470 = t50.*t202.*(t4699-t5039-t5041+t5048-t5049+t3880.*(t2694-t2701+t3036-t3043).*1.6e-7+t3901.*(-t1881+t3121+t3269).*1.6e-7+t3901.*(-t1901+t3122+t3270).*5.0e-8);
et471 = 5.673626844500105e-17;
et472 = t4987+t5332-t5615-t5835-t5876+t5879-t5958+t5970+t6323+t6529-t6701-t6860+t6861+t6954+t7204+t7219+t7505+t7952-t244.*(t4173+t4965+t123.*t188.*(t2694-t2701+t3036-t3043).*2.442490654175345e-23+t50.*t189.*t4860.*(t42-t43).*2.711709361697228e-39);
et473 = t3385.*(t5453-t5460+t5543+t5544-t5550-t5556+t4865.*(t3951+t18.*(t1861-t3214)).*9.3e-7+t4860.*(t3493-t3972).*9.0e-8)+t2363.*(et468+et469)+t6617.*(t2527-t3009);
et474 = t3901.*t4175.*(t1554+t2361+t2362+t2367+t2414+t3928+t3934+t4160+t4163+t17.*(-t1901+t3122+t3270).*5.68686e-3).*1.08769e-2+t3498.*t5150.*(t2694-t2701+t3036-t3043).*2.889644e-2+t3628.*t5509.*(t2694-t2701+t3036-t3043).*2.889644e-2;
et475 = t3910.*t5426.*(t2694-t2701+t3036-t3043).*1.08769e-2+t4304.*t5798.*(t2694-t2701+t3036-t3043).*7.26735e-3-t3498.*t3901.*(-t56+t60+t649+t670+t686+t687+t1577+t1578+t1586+t1600+t2303+t2339+t2689+t3030+t3292+t3305).*2.889644e-2;
et476 = t3628.*t4860.*(-t56+t60+t649+t670+t686+t687+t1577+t1578+t1586+t1600+t2303+t2339+t2689+t3030+t3292+t3305).*(-2.889644e-2)+t3901.*t3910.*t5437.*1.08769e-2-t3628.*t4865.*t5150.*2.889644e-2+t3901.*t4304.*t5800.*7.26735e-3;
et477 = t4175.*t4865.*t5426.*1.08769e-2-t4175.*t4860.*t5437.*1.08769e-2-t4860.*t5800.*(t1513+t1879+t2598+t2820+t2834+t3117+t3118).*7.26735e-3+t4865.*t5798.*(t1513+t1879+t2598+t2820+t2834+t3117+t3118).*7.26735e-3+et470.*et471;
et478 = t6345+t7292+t4824.*(t4737+t4744+t4751+t3942.*(t2694-t2701+t3036-t3043).*5.7e-7)+t3996.*(t5231+t5235-t5273+t5278+t5282-t5285+t4777.*(t2694-t2701+t3036-t3043).*5.7e-7+t4780.*(t2694-t2701+t3036-t3043).*4.0e-8);
et479 = t3992.*(-t5152+t5230+t5241+t5276-t5277-t5281+t5286+(t4865.*(t1861-t3214))./1.0e+8+(t3901.*(t951+t16.*(-t1881+t3121+t3269)))./1.0e+8+(t4080.*(t2694-t2701+t3036-t3043))./1.0e+8+t4777.*(t2694-t2701+t3036-t3043).*4.0e-8+t4780.*(t2694-t2701+t3036-t3043).*2.4e-7);
et480 = t4814.*(-t4437-t4438+t4741+t4767+t3942.*(t2694-t2701+t3036-t3043).*4.0e-8+t3946.*(t2694-t2701+t3036-t3043).*2.4e-7);
et481 = t237.*6.47e-6;
et482 = t238.*5.84482e-3-t50.*t189.*3.311325901843639e-18;
et483 = t16.*t50.*t189.*3.31613276532711e-19-t21.*t50.*t189.*3.670836568391568e-22;
et484 = -t2306-t2317+t3144+t3147+t35.*t941.*t948.*(t850-t874).*3.775747223193135e-1;
et485 = t36.*t941.*t948.*(t850-t874).*2.244797987218524e-1;
et486 = t3230.*(t4686-t5035+t5038-t5040-t5047+t3880.*(t2694-t2701+t3036-t3043).*5.0e-8+t3901.*(-t1881+t3121+t3269).*5.0e-8+t3901.*(-t1901+t3122+t3270).*1.1e-7)-t3898.*t5853-t3904.*t5852;
et487 = t3231.*(t4699-t5039-t5041+t5048-t5049+t3880.*(t2694-t2701+t3036-t3043).*1.6e-7+t3901.*(-t1881+t3121+t3269).*1.6e-7+t3901.*(-t1901+t3122+t3270).*5.0e-8)+(t201.*t4977.*(t46-t47))./9.007199254740992e+15;
et488 = t50.*t202.*(t46-t47).*(t4173+t4965+t123.*t188.*(t2694-t2701+t3036-t3043).*2.442490654175345e-23+t50.*t189.*t4860.*(t42-t43).*2.711709361697228e-39).*(-1.232595164407831e-32);
et489 = t262.*1.869599668e-7;
et490 = t264.*1.688944904408e-4;
et491 = t50.*t202.*(-9.568553024307061e-20);
et492 = t26.*t50.*t202.*9.582443148530891e-21;
et493 = t32.*t50.*t202.*(-1.060741086483328e-23);
et494 = -t2306-t2317+t3144+t3147+t35.*t941.*t948.*(t850-t874).*3.775747223193135e-1;
et495 = t36.*t941.*t948.*(t850-t874).*2.244797987218524e-1;
et496 = t3229.*(t4686-t5035+t5038-t5040-t5047+t3880.*(t2694-t2701+t3036-t3043).*5.0e-8+t3901.*(-t1881+t3121+t3269).*5.0e-8+t3901.*(-t1901+t3122+t3270).*1.1e-7);
et497 = t5853.*(t1941-t3308+t39.*t1022.*(t855-t878).*2.196325630278387e-1)-t5852.*(t1959-t3306+t38.*t1022.*(t855-t878).*2.196325630278387e-1);
et498 = -t3228.*(t4699-t5039-t5041+t5048-t5049+t3880.*(t2694-t2701+t3036-t3043).*1.6e-7+t3901.*(-t1881+t3121+t3269).*1.6e-7+t3901.*(-t1901+t3122+t3270).*5.0e-8)-(t140.*t201.*t4977)./9.007199254740992e+15;
et499 = (t50.*t140.*t202.*(t4173+t4965+t123.*t188.*(t2694-t2701+t3036-t3043).*2.442490654175345e-23+t50.*t189.*t4860.*(t42-t43).*2.711709361697228e-39))./8.112963841460668e+31;
et500 = -t2306-t2317+t3144+t3147+t35.*t941.*t948.*(t850-t874).*3.775747223193135e-1;
et501 = t36.*t941.*t948.*(t850-t874).*2.244797987218524e-1;
et502 = -t2306-t2317+t3144+t3147+t35.*t941.*t948.*(t850-t874).*3.775747223193135e-1;
et503 = t36.*t941.*t948.*(t850-t874).*2.244797987218524e-1;
et504 = -t2306-t2317+t3144+t3147+t35.*t941.*t948.*(t850-t874).*3.775747223193135e-1;
et505 = t36.*t941.*t948.*(t850-t874).*2.244797987218524e-1;
et506 = -t2306-t2317+t3144+t3147+t35.*t941.*t948.*(t850-t874).*3.775747223193135e-1;
et507 = t36.*t941.*t948.*(t850-t874).*2.244797987218524e-1;
et508 = -t2306-t2317+t3144+t3147+t35.*t941.*t948.*(t850-t874).*3.775747223193135e-1;
et509 = t36.*t941.*t948.*(t850-t874).*2.244797987218524e-1;
et510 = -t3877.*(et478+et479+et480)+t4822.*(t6887+t3985.*(t4737+t4744+t4751+t3942.*(t2694-t2701+t3036-t3043).*5.7e-7)+t6088.*(t1896-t3232))-t3974.*t4444-t4279.*t4281-t3877.*t7790-t3877.*t7954+t4822.*t7440+t3783.*(et481+et482+et483);
et511 = (t6214+t3996.*(t4737+t4744+t4751+t3942.*(t2694-t2701+t3036-t3043).*5.7e-7)+t3992.*(-t4437-t4438+t4741+t4767+t3942.*(t2694-t2701+t3036-t3043).*4.0e-8+t3946.*(t2694-t2701+t3036-t3043).*2.4e-7)).*(et484+et485)+t3877.*(et486+et487+et488)+t3480.*(et489+et490+et491+et492+et493);
et512 = (t3230.*t5852+t3231.*t5853+(t50.*t202.*t4977.*(t46-t47))./8.112963841460668e+31).*(et494+et495)+(t2674-t2676+t3022-t3027).*(et496+et497+et498+et499);
et513 = -(t2674-t2676+t3022-t3027).*(t6993+t7293+t7349+t7566-t6088.*(t1005+t26.*(t1941-t3308+t39.*t1022.*(t855-t878).*2.196325630278387e-1))-t4817.*(t4737+t4744+t4751+t3942.*(t2694-t2701+t3036-t3043).*5.7e-7));
et514 = -t4822.*(t3228.*t5853-t3229.*t5852+(t50.*t140.*t202.*t4977)./8.112963841460668e+31)+t7791.*(t2674-t2676+t3022-t3027)+t7953.*(t2674-t2676+t3022-t3027)+t7181.*(et500+et501)+t7443.*(et502+et503)+t4822.*(-t5468+t5998+t5943.*(t1896-t3232))+t3901.*(et504+et505).*(t1488+t1874+t2519+t2740+t2747+t3096+t3097).*(t1513+t1879+t2598+t2820+t2834+t3117+t3118).*7.26735e-3;
et515 = t3480.*t3628.*(t2674-t2676+t3022-t3027).*(t2694-t2701+t3036-t3043).*(-2.889644e-2)-t3498.*t3617.*(t2674-t2676+t3022-t3027).*(t2694-t2701+t3036-t3043).*2.889644e-2+t3910.*t4134.*(t2674-t2676+t3022-t3027).*(t2694-t2701+t3036-t3043).*1.08769e-2;
et516 = t3891.*t4175.*(t2674-t2676+t3022-t3027).*(t2694-t2701+t3036-t3043).*1.08769e-2+t236.*t241.*t4500.*t4655.*4.312975891071717e-75;
et517 = t236.*t241.*t4589.*t4644.*(-4.312975891071717e-75)-t3480.*t3628.*t3877.*t3901.*2.889644e-2-t3498.*t3617.*t3877.*t3901.*2.889644e-2;
et518 = t3877.*t3901.*t3910.*t4134.*1.08769e-2+t3877.*t3891.*t3901.*t4175.*1.08769e-2-t3617.*t3628.*t3877.*t4860.*2.889644e-2-t3877.*t4134.*t4175.*t4860.*1.08769e-2;
et519 = t4304.*(t2674-t2676+t3022-t3027).*(t2694-t2701+t3036-t3043).*(t1488+t1874+t2519+t2740+t2747+t3096+t3097).*7.26735e-3+t4298.*(t2674-t2676+t3022-t3027).*(t2694-t2701+t3036-t3043).*(t1513+t1879+t2598+t2820+t2834+t3117+t3118).*7.26735e-3+t3877.*t3901.*t4304.*(t1488+t1874+t2519+t2740+t2747+t3096+t3097).*7.26735e-3;
et520 = t3877.*t3901.*t4298.*(t1513+t1879+t2598+t2820+t2834+t3117+t3118).*7.26735e-3-t3877.*t4860.*(t1488+t1874+t2519+t2740+t2747+t3096+t3097).*(t1513+t1879+t2598+t2820+t2834+t3117+t3118).*7.26735e-3+t3617.*t3628.*t4865.*(t2674-t2676+t3022-t3027).*2.889644e-2;
et521 = t3617.*t3628.*t4822.*(t2694-t2701+t3036-t3043).*2.889644e-2+t4134.*t4175.*t4865.*(t2674-t2676+t3022-t3027).*1.08769e-2+t4134.*t4175.*t4822.*(t2694-t2701+t3036-t3043).*1.08769e-2;
et522 = t4865.*(t2674-t2676+t3022-t3027).*(t1488+t1874+t2519+t2740+t2747+t3096+t3097).*(t1513+t1879+t2598+t2820+t2834+t3117+t3118).*7.26735e-3+t4822.*(t2694-t2701+t3036-t3043).*(t1488+t1874+t2519+t2740+t2747+t3096+t3097).*(t1513+t1879+t2598+t2820+t2834+t3117+t3118).*7.26735e-3+t3617.*t3628.*t3901.*(et506+et507).*2.889644e-2;
et523 = t3901.*t4134.*t4175.*(et508+et509).*1.08769e-2;
et524 = t4688-t5036+t5042-t5164+t4865.*(t1861-t3214).*7.83e-6+t3901.*(t951+t16.*(-t1881+t3121+t3269)).*7.83e-6+t4080.*(t2694-t2701+t3036-t3043).*7.83e-6;
et525 = t3901.*(-t1901+t3122+t3270).*3.24e-6;
et526 = t50.*t202.*(t4699-t5039-t5041+t5048-t5049+t3880.*(t2694-t2701+t3036-t3043).*1.6e-7+t3901.*(-t1881+t3121+t3269).*1.6e-7+t3901.*(-t1901+t3122+t3270).*5.0e-8);
et527 = 5.673626844500105e-17;
et528 = t4987+t5332-t5615-t5835-t5876+t5879-t5958+t5970+t6323+t6529-t6701-t6860+t6861+t6954+t7204+t7219+t7505+t7952-t244.*(t4173+t4965+t123.*t188.*(t2694-t2701+t3036-t3043).*2.442490654175345e-23+t50.*t189.*t4860.*(t42-t43).*2.711709361697228e-39);
et529 = t3385.*(t5453-t5460+t5543+t5544-t5550-t5556+t4865.*(t3951+t18.*(t1861-t3214)).*9.3e-7+t4860.*(t3493-t3972).*9.0e-8)+t2363.*(et524+et525)+t6617.*(t2527-t3009);
et530 = t3901.*t4175.*(t1554+t2361+t2362+t2367+t2414+t3928+t3934+t4160+t4163+t17.*(-t1901+t3122+t3270).*5.68686e-3).*1.08769e-2+t3498.*t5151.*(t2694-t2701+t3036-t3043).*2.889644e-2+t3628.*t5509.*(t2694-t2701+t3036-t3043).*2.889644e-2;
et531 = t3910.*t5429.*(t2694-t2701+t3036-t3043).*1.08769e-2+t4304.*t5799.*(t2694-t2701+t3036-t3043).*7.26735e-3-t3498.*t3901.*t5155.*2.889644e-2-t3628.*t4860.*t5155.*2.889644e-2;
et532 = t3628.*t4865.*t5151.*(-2.889644e-2)+t3901.*t4304.*t5801.*7.26735e-3+t4175.*t4865.*t5429.*1.08769e-2-t4860.*t5801.*(t1513+t1879+t2598+t2820+t2834+t3117+t3118).*7.26735e-3;
et533 = t4865.*t5799.*(t1513+t1879+t2598+t2820+t2834+t3117+t3118).*7.26735e-3+et526.*et527-t3901.*t3910.*(t410-t5413).*1.08769e-2+t4175.*t4860.*(t410-t5413).*1.08769e-2;
et534 = t6345+t7292+t4824.*(t4737+t4744+t4751+t3942.*(t2694-t2701+t3036-t3043).*5.7e-7)+t3996.*(t5231+t5235-t5273+t5278+t5282-t5285+t4777.*(t2694-t2701+t3036-t3043).*5.7e-7+t4780.*(t2694-t2701+t3036-t3043).*4.0e-8);
et535 = t3992.*(-t5152+t5230+t5241+t5276-t5277-t5281+t5286+(t4865.*(t1861-t3214))./1.0e+8+(t3901.*(t951+t16.*(-t1881+t3121+t3269)))./1.0e+8+(t4080.*(t2694-t2701+t3036-t3043))./1.0e+8+t4777.*(t2694-t2701+t3036-t3043).*4.0e-8+t4780.*(t2694-t2701+t3036-t3043).*2.4e-7);
et536 = t4814.*(-t4437-t4438+t4741+t4767+t3942.*(t2694-t2701+t3036-t3043).*4.0e-8+t3946.*(t2694-t2701+t3036-t3043).*2.4e-7);
et537 = t707+t708-t721-t722-t749+t762+t768-t777-t792-t793-t801-t802-t808+t813-t819+t821-t1629+t1637-t1640-t1641-t1659-t1661+t1666+t1667+t1683+t1692+t1705-t1712+t1758+t1759+t1775+t1776+t1973+t1993+t1994+t2023+t2053+t2060-t2089-t2090+t2098+t2099-t14.*t15.*t21.*t50.*t189.*3.670836568391568e-22;
et538 = t16.*t19.*t20.*t50.*t189.*(-3.279367663374749e-19)-t14.*t15.*t17.*t21.*t50.*t189.*7.075931802640439e-19;
et539 = t14.*t17.*t20.*t21.*t50.*t189.*(-1.190170786299927e-18)-t15.*t17.*t19.*t21.*t50.*t189.*1.190170786299927e-18;
et540 = t19.*t20.*t21.*t22.*t50.*t189.*(-3.226512155691387e-19);
et541 = t707+t708-t721-t722-t749+t762+t768-t777-t792-t793-t801-t802-t808+t813-t819+t821-t1629+t1637-t1640-t1641-t1659-t1661+t1666+t1667+t1683+t1692+t1705-t1712+t1758+t1759+t1775+t1776+t1973+t1993+t1994+t2023+t2053+t2060-t2089-t2090+t2098+t2099-t14.*t15.*t21.*t50.*t189.*3.670836568391568e-22;
et542 = t16.*t19.*t20.*t50.*t189.*(-3.279367663374749e-19)-t14.*t15.*t17.*t21.*t50.*t189.*7.075931802640439e-19;
et543 = t14.*t17.*t20.*t21.*t50.*t189.*(-1.190170786299927e-18)-t15.*t17.*t19.*t21.*t50.*t189.*1.190170786299927e-18;
et544 = t19.*t20.*t21.*t22.*t50.*t189.*(-3.226512155691387e-19);
et545 = t4688-t5036+t5042-t5164+t4865.*(t1861-t3214).*7.83e-6+t3901.*(t951+t16.*(-t1881+t3121+t3269)).*7.83e-6+t4080.*(t2694-t2701+t3036-t3043).*7.83e-6;
et546 = t3901.*(-t1901+t3122+t3270).*3.24e-6;
et547 = -t3210.*(et534+et535+et536)-t3209.*(t6993+t7293+t7349+t7566-t6088.*(t1005+t26.*(t1941-t3308+t39.*t1022.*(t855-t878).*2.196325630278387e-1))-t4817.*(t4737+t4744+t4751+t3942.*(t2694-t2701+t3036-t3043).*5.7e-7));
et548 = t188.*(t2388.*t5291-t2363.*t5943+t50.*t202.*t5944.*9.543032792050485e-17).*8.595599785252598e-1-t3882.*(t6887+t3985.*(t4737+t4744+t4751+t3942.*(t2694-t2701+t3036-t3043).*5.7e-7)+t6088.*(t1896-t3232));
et549 = t188.*t7352.*8.595599785252598e-1-t3871.*t4279+t3869.*t4444+t3209.*t7791-t3210.*t7790+t3209.*t7953-t3210.*t7954-t3882.*t7440;
et550 = (-t1901+t3122+t3270).*(t6214+t3996.*(t4737+t4744+t4751+t3942.*(t2694-t2701+t3036-t3043).*5.7e-7)+t3992.*(-t4437-t4438+t4741+t4767+t3942.*(t2694-t2701+t3036-t3043).*4.0e-8+t3946.*(t2694-t2701+t3036-t3043).*2.4e-7));
et551 = t188.*(-t6123+t6359+t3057.*(-t4437-t4438+t4741+t4767+t3942.*(t2694-t2701+t3036-t3043).*4.0e-8+t3946.*(t2694-t2701+t3036-t3043).*2.4e-7)).*8.595599785252598e-1+t7181.*(-t1901+t3122+t3270)+t7443.*(-t1901+t3122+t3270)-t3882.*(-t5468+t5998+t5943.*(t1896-t3232));
et552 = t3910.*t5951.*(t2694-t2701+t3036-t3043).*1.08769e-2-t4175.*t5722.*(t2694-t2701+t3036-t3043).*1.08769e-2+t4304.*t6561.*(t2694-t2701+t3036-t3043).*7.26735e-3;
et553 = t7353.*(t2694-t2701+t3036-t3043).*(t1513+t1879+t2598+t2820+t2834+t3117+t3118).*7.26735e-3+t3901.*t3910.*(et537+et538+et539+et540).*1.08769e-2-t4175.*t4860.*(et541+et542+et543+et544).*1.08769e-2;
et554 = t50.*t189.*(t5332-t5958+t5970+t6529+t7219+t2363.*(et545+et546)).*(-9.543032792050485e-17)+t50.*t189.*t7931.*9.543032792050485e-17-t50.*t189.*t7952.*9.543032792050485e-17;
et555 = t3901.*t4175.*t5723.*(-1.08769e-2)+t3901.*t4304.*t6564.*7.26735e-3+t4175.*t4865.*t5951.*1.08769e-2+t3901.*t7354.*(t1513+t1879+t2598+t2820+t2834+t3117+t3118).*7.26735e-3;
et556 = t4860.*t6564.*(t1513+t1879+t2598+t2820+t2834+t3117+t3118).*(-7.26735e-3)+t4865.*t6561.*(t1513+t1879+t2598+t2820+t2834+t3117+t3118).*7.26735e-3;
et557 = t236.*t241.*t4620.*t4655.*2.33806891548878e-94;
et558 = t236.*t241.*t4589.*t4974.*(-2.33806891548878e-94);
et559 = -t5289-t5516-t5900+t5923-t6169+t6294-t6942+t7200+t7202-t7262+t7521+t7525;
et560 = t4080.*(t4510.*(t2813-t2835+t18.*(t1456-t2355).*1.02e-6+t23.*(t1456-t2355).*9.0e-8)+t4514.*(-t2804+t2838+t3109+t23.*(t1456-t2355).*9.3e-7)+t3132.*(t3235-t3535));
et561 = t6565.*(t4758.*(t1861-t3214)+t2297.*(t642+t643-t667+t674+t1587+t1606+t1608+t1609+t2295+t2671+t2683+t2684-t2695+t3272+t3290-t3296+t3576+t3582+t3588-t3593+t4015+t4016))+t5756.*(t951+t16.*(-t1881+t3121+t3269))+(t1861-t3214).*(t4595+t4658+t5189+t5207-t3468.*(t1005+t26.*(t1941-t3308+t39.*t1022.*(t855-t878).*2.196325630278387e-1))-t3420.*(t1896-t3232));
et562 = -t2306-t2317+t3144+t3147+t35.*t941.*t948.*(t850-t874).*3.775747223193135e-1;
et563 = t36.*t941.*t948.*(t850-t874).*2.244797987218524e-1;
et564 = -t2306-t2317+t3144+t3147+t35.*t941.*t948.*(t850-t874).*3.775747223193135e-1;
et565 = t36.*t941.*t948.*(t850-t874).*2.244797987218524e-1;
et566 = -t2306-t2317+t3144+t3147+t35.*t941.*t948.*(t850-t874).*3.775747223193135e-1;
et567 = t36.*t941.*t948.*(t850-t874).*2.244797987218524e-1;
et568 = t4219+t4242+t4663+t4702-t5245-t5246-t5247-t5248+t5345+t5348-t5433-t5434-t5440-t5441+t7295-t7297+t7776-t7782+t3877.*(t5582+t5715-t6598-t6801+t6802+t6413.*(t3544-t4013))+t7757.*(t2674-t2676+t3022-t3027)+t3984.*(t2674-t2676+t3022-t3027).*(t2694-t2701+t3036-t3043).*(t1488+t1874+t2519+t2740+t2747+t3096+t3097).*7.26735e-3;
et569 = t3941.*(t2674-t2676+t3022-t3027).*(t2694-t2701+t3036-t3043).*(t1513+t1879+t2598+t2820+t2834+t3117+t3118).*7.26735e-3+t3877.*t3901.*t3984.*(t1488+t1874+t2519+t2740+t2747+t3096+t3097).*7.26735e-3+t3877.*t3901.*t3941.*(t1513+t1879+t2598+t2820+t2834+t3117+t3118).*7.26735e-3;
et570 = -t5196-t5322-t5330+t5331+t5335+t5504+t5506+t5558+t5810-t5969+t6113-t6117+t7693+t7735+(t2694-t2701+t3036-t3043).*(t3505.*1.838876e-2-t3570+t3571+t22.*(t1861-t3214).*(3.0./5.0e+2)+t22.*t23.*(t1861-t3214).*9.99471e-3).*(t1513+t1879+t2598+t2820+t2834+t3117+t3118).*7.26735e-3;
et571 = t3628.*t4277.*(t2694-t2701+t3036-t3043).*2.889644e-2+t3732.*t5426.*(t2694-t2701+t3036-t3043).*1.08769e-2+t3359.*t3901.*(-t56+t60+t649+t670+t686+t687+t1577+t1578+t1586+t1600+t2303+t2339+t2689+t3030+t3292+t3305).*2.889644e-2;
et572 = t3901.*t5220.*(t1513+t1879+t2598+t2820+t2834+t3117+t3118).*7.26735e-3;
et573 = t1288+t1289+t1302+t1303-t1319-t1320+t1336-t1348+t1350+t1351-t1360+t1369-t1378+t1396-t1425+t1435-t2174+t2183-t2187+t2193-t2194-t2195+t2199-t2203-t2215+t2219-t2222-t2223+t2239+t2240-t2256-t2257+t2555+t2556+t2572+t2583-t2605-t2606+t2612+t2613-t2618-t2619+t2651+t2652;
et574 = t24.*t25.*t26.*t50.*t202.*(-3.566935413776081e-21);
et575 = t30.*t31.*t32.*t50.*t202.*(-3.992732227073824e-24);
et576 = t24.*t25.*t32.*t33.*t50.*t202.*(-3.509445006623964e-21);
et577 = t27.*t30.*t31.*t32.*t50.*t202.*(-7.696420262413979e-21);
et578 = (t4.*(-t4911+t5005-t5488+t5578-t6206+t6207+t6508+t6689-t6692+t6940+t7086+t7359+t7424+t7444+t7446-t7733-t7734-t7897-t7898+t7917-t7919+t4822.*(-t5209+t5751+t5639.*(t1896-t3232))+t6975.*(et562+et563)+t7326.*(et564+et565)+t7363.*(et566+et567)+t3891.*t6183.*(t2674-t2676+t3022-t3027)+t4298.*t6595.*(t2674-t2676+t3022-t3027)+t4822.*t6595.*(t1488+t1874+t2519+t2740+t2747+t3096+t3097)))./2.0-t4.*(et568+et569)-t2.*(et570+et571+et572);
et579 = (t5.*(t4868+t4869-t5620+t5626+t6809-t6811+t6812-t6892+t7054+t7299+t7319-t7336-t7389+t7579+t7581+t7583-t7665-t7730+t7731+t7854+t7865+t7892-t7894-t7910-t7911+t5723.*(et573+et574+et575+et576+et577)+t6564.*(t4983-t5225-t6233+t7058)+t6975.*(-t1901+t3122+t3270)+t7326.*(-t1901+t3122+t3270)+t7363.*(-t1901+t3122+t3270)))./2.0+(t2.*t8035)./2.0+(t3.*t8036)./2.0+t5.*t8040-t6.*t8045+(t6.*t8049)./2.0;
et580 = (t7.*(t7322-t7422+t7871-t7920-t7921+t7363.*(t17.*((t237.*(t42-t43))./9.007199254740992e+15+t21.*(-t1881+t3121+t3269))+t22.*(-t1901+t3122+t3270))))./2.0-t7.*(-t7356+t7466+t7700-t7779+t3957.*(t5582+t5715-t6598-t6801+t6802+t6413.*(t3544-t4013))+t17.*t7440.*(t1861-t3214));
et581 = t3.*(t5196+t5322+t5330-t5331-t5335-t5365+t5505+t5507+t5561+t5575+t5585+t5809+t5813+t5832+t5833+t5969+t5997+t6020+t6116+t6118+t6124+t6348+t6477+t6478+t6534+t6697+t6698+t6777-t3628.*t4277.*(t2694-t2701+t3036-t3043).*2.889644e-2);
et582 = t5338+t5340+t7725-t7727+t4149.*(t2674-t2676+t3022-t3027).*(t2694-t2701+t3036-t3043).*(t1488+t1874+t2519+t2740+t2747+t3096+t3097).*7.26735e-3+t4108.*(t2674-t2676+t3022-t3027).*(t2694-t2701+t3036-t3043).*(t1513+t1879+t2598+t2820+t2834+t3117+t3118).*7.26735e-3+t3877.*t3901.*t4149.*(t1488+t1874+t2519+t2740+t2747+t3096+t3097).*7.26735e-3;
et583 = t3877.*t3901.*t4108.*(t1513+t1879+t2598+t2820+t2834+t3117+t3118).*7.26735e-3;
et584 = -t2306-t2317+t3144+t3147+t35.*t941.*t948.*(t850-t874).*3.775747223193135e-1;
et585 = t36.*t941.*t948.*(t850-t874).*2.244797987218524e-1;
et586 = -t5289-t5516-t5900+t5923-t6169+t6294-t6942+t7200+t7202-t7262+t7523+t7527;
et587 = t4080.*(t4510.*(t2813-t2835+t18.*(t1456-t2355).*1.02e-6+t23.*(t1456-t2355).*9.0e-8)+t4514.*(-t2804+t2838+t3109+t23.*(t1456-t2355).*9.3e-7)+t3132.*(t3235-t3535));
et588 = t6565.*(t4758.*(t1861-t3214)+t2297.*(t642+t643-t667+t674+t1587+t1606+t1608+t1609+t2295+t2671+t2683+t2684-t2695+t3272+t3290-t3296+t3576+t3582+t3588-t3593+t4015+t4016))+t5756.*(t951+t16.*(-t1881+t3121+t3269))+(t1861-t3214).*(t4595+t4658+t5189+t5207-t3468.*(t1005+t26.*(t1941-t3308+t39.*t1022.*(t855-t878).*2.196325630278387e-1))-t3420.*(t1896-t3232));
et589 = -t6.*(et454+et455+et456)+t4.*((t6.*(et460+et461+et462+et463+et464+et465+et466+et467))./2.0-(t2.*(et472+et473+et474+et475+et476+et477))./2.0+(t4.*(et510+et511+et512+et513+et514+et515+et516+et517+et518+et519+et520+et521+et522+et523))./2.0+(t7.*(t2994.*t7352+t3047.*t7931+t3946.*t7953-t3957.*t7954-t4780.*t7440+t7443.*(t17.*((t237.*(t42-t43))./9.007199254740992e+15+t21.*(-t1881+t3121+t3269))+t22.*(-t1901+t3122+t3270))))./2.0-(t3.*(et528+et529+et530+et531+et532+et533))./2.0+(t5.*(et547+et548+et549+et550+et551+et552+et553+et554+et555+et556+et557+et558))./2.0);
et590 = -t2.*(t7789-(t2.*t7992)./2.0-(t3.*t7991)./2.0+(t4.*t8019)./2.0+(t5.*t8021)./2.0-(t6.*(et559+et560+et561))./2.0)-t5.*(et578+et579+et580+et581);
et591 = -t7.*((t5.*(t7492-t7554+t7956+t7968-t7970+t7540.*(-t1901+t3122+t3270)))./2.0-t2.*t7796-t3.*t7797+(t2.*t7955)./2.0+(t3.*t7955)./2.0+t7.*t7985-t5.*t8001-t6.*t8002+(t6.*t8042)./2.0+(t4.*(t7570-t7973-t7974+t7540.*(et584+et585)))./2.0+(t7.*(t7498-t7568+t7959+t7975-t7977+t7540.*(t17.*((t237.*(t42-t43))./9.007199254740992e+15+t21.*(-t1881+t3121+t3269))+t22.*(-t1901+t3122+t3270))))./2.0-t4.*(et582+et583));
et592 = -t3.*(t7789-(t2.*t7990)./2.0-(t3.*t7989)./2.0+(t4.*t8020)./2.0+(t5.*t8022)./2.0-(t6.*(et586+et587+et588))./2.0+t2.*(t5595+t5601-t5617-t5619-t5858+t5873+t5885+t6223+t6229-t6256+t4175.*t5413.*(t2694-t2701+t3036-t3043).*1.08769e-2+t3901.*t5798.*(t1513+t1879+t2598+t2820+t2834+t3117+t3118).*7.26735e-3));
et593 = t2297.*(-t5400+t6300-t6540+t6541+t3385.*(t3417-t3421-t4507+t4513+t4519-t4540)+t3057.*(-t3080+t4062+t17.*t3229.*(t1861-t3214).*1.02e-6))+t3483.*(t5357-t5512+t6671-t6674+t4541.*(t3417-t3421-t4507+t4513+t4519-t4540)+t6172.*(t3544-t4013))+t2307.*t7298+t2307.*t7318+t2297.*t7615-t3481.*t7325+t3484.*t7326-t3481.*t7362+t3484.*t7363-t3483.*t7638+t6005.*t6631;
et594 = t6002.*(t4758.*(t1861-t3214)+t2297.*(t642+t643-t667+t674+t1587+t1606+t1608+t1609+t2295+t2671+t2683+t2684-t2695+t3272+t3290-t3296+t3576+t3582+t3588-t3593+t4015+t4016))+t7637.*(t1861-t3214)-t7678.*(t1861-t3214);
et595 = t6595.*(t4785+t5058+t2307.*(t642+t643-t667+t674+t1587+t1606+t1608+t1609+t2295+t2671+t2683+t2684-t2695+t3272+t3290-t3296+t3576+t3582+t3588-t3593+t4015+t4016)+t2297.*(t2292+t3283+t3505.*1.838876e-2-t3570+t3571+t3590+t22.*(t1861-t3214).*3.131399999999998e-4+t22.*t23.*(t1861-t3214).*9.99471e-3))-t6606.*(t4786+t5069-t5665-t6291);
et596 = t236.*t241.*t4280.*t4985.*2.595777943136013e-110;
et597 = t236.*t241.*t4705.*t4986.*(-2.595777943136013e-110);
et598 = t707+t708-t721-t722-t749+t762+t768-t777-t792-t793-t801-t802-t808+t813-t819+t821-t1629+t1637-t1640-t1641-t1659-t1661+t1666+t1667+t1683+t1692+t1705-t1712+t1758+t1759+t1775+t1776+t1973+t1993+t1994+t2023+t2053+t2060-t2089-t2090+t2098+t2099-t14.*t15.*t21.*t50.*t189.*3.670836568391568e-22;
et599 = t16.*t19.*t20.*t50.*t189.*(-3.279367663374749e-19)-t14.*t15.*t17.*t21.*t50.*t189.*7.075931802640439e-19;
et600 = t14.*t17.*t20.*t21.*t50.*t189.*(-1.190170786299927e-18)-t15.*t17.*t19.*t21.*t50.*t189.*1.190170786299927e-18;
et601 = t19.*t20.*t21.*t22.*t50.*t189.*(-3.226512155691387e-19);
et602 = t1288+t1289+t1302+t1303-t1319-t1320+t1336-t1348+t1350+t1351-t1360+t1369-t1378+t1396-t1425+t1435-t2174+t2183-t2187+t2193-t2194-t2195+t2199-t2203-t2215+t2219-t2222-t2223+t2239+t2240-t2256-t2257+t2555+t2556+t2572+t2583-t2605-t2606+t2612+t2613-t2618-t2619+t2651+t2652;
et603 = t24.*t25.*t26.*t50.*t202.*(-3.566935413776081e-21);
et604 = t30.*t31.*t32.*t50.*t202.*(-3.992732227073824e-24);
et605 = t24.*t25.*t32.*t33.*t50.*t202.*(-3.509445006623964e-21);
et606 = t27.*t30.*t31.*t32.*t50.*t202.*(-7.696420262413979e-21);
et607 = -t6185.*(et598+et599+et600+et601)-t3210.*(t5357-t5512+t6671-t6674+t4541.*(t3417-t3421-t4507+t4513+t4519-t4540)+t6172.*(t3544-t4013))+t3869.*t4230+t3870.*t4231-t3210.*t7179-t3209.*t7637+t3210.*t7638+t3209.*t7678-t5951.*t6184-t5953.*t6183+t6002.*t6561+t6005.*t6564+t5975.*t6595+t5976.*t6606+t5954.*(et602+et603+et604+et605+et606)-t3209.*(t5192+t5210-t5765+t3524.*(-t3064+t4027+t3229.*(t1861-t3214).*9.840000000000001e-6)+t4992.*(t1896-t3232));
et608 = t50.*t189.*(-t5400+t6300-t6540+t6541+t3385.*(t3417-t3421-t4507+t4513+t4519-t4540)+t3057.*(-t3080+t4062+t17.*t3229.*(t1861-t3214).*1.02e-6)).*9.543032792050485e-17+t50.*t189.*t7615.*9.543032792050485e-17;
et609 = t50.*t189.*(t5034+t5051+t5052+t5057+t5689).*(-9.543032792050485e-17);
et610 = t236.*t241.*t4974.*t4986.*1.267469698796881e-113;
et611 = t236.*t241.*t4976.*t4985.*1.267469698796881e-113;
et612 = t1288+t1289+t1302+t1303-t1319-t1320+t1336-t1348+t1350+t1351-t1360+t1369-t1378+t1396-t1425+t1435-t2174+t2183-t2187+t2193-t2194-t2195+t2199-t2203-t2215+t2219-t2222-t2223+t2239+t2240-t2256-t2257+t2555+t2556+t2572+t2583-t2605-t2606+t2612+t2613-t2618-t2619+t2651+t2652;
et613 = t24.*t25.*t26.*t50.*t202.*(-3.566935413776081e-21);
et614 = t30.*t31.*t32.*t50.*t202.*(-3.992732227073824e-24);
et615 = t24.*t25.*t32.*t33.*t50.*t202.*(-3.509445006623964e-21);
et616 = t27.*t30.*t31.*t32.*t50.*t202.*(-7.696420262413979e-21);
et617 = (t2674-t2676+t3022-t3027).*(t5192+t5210-t5765+t3524.*(-t3064+t4027+t3229.*(t1861-t3214).*9.840000000000001e-6)+t4992.*(t1896-t3232))+t3877.*(t5357-t5512+t6671-t6674+t4541.*(t3417-t3421-t4507+t4513+t4519-t4540)+t6172.*(t3544-t4013))+t3779.*t4231+t3974.*t4230+t3877.*t7179-t3877.*t7638+t7637.*(t2674-t2676+t3022-t3027)-t7678.*(t2674-t2676+t3022-t3027)+t3689.*t6183.*(t2674-t2676+t3022-t3027)+t4134.*t6184.*(t2674-t2676+t3022-t3027);
et618 = -t3941.*t6595.*(t2674-t2676+t3022-t3027)-t6002.*(t2674-t2676+t3022-t3027).*(t1488+t1874+t2519+t2740+t2747+t3096+t3097)+t3877.*t4134.*t6185-t3877.*t3941.*t6606-t3877.*t6005.*(t1488+t1874+t2519+t2740+t2747+t3096+t3097)-t3689.*t3877.*(et612+et613+et614+et615+et616);
et619 = t236.*t241.*t4295.*t4985.*(-2.33806891548878e-94);
et620 = t236.*t241.*t4644.*t4986.*(-2.33806891548878e-94);
et621 = -t5034-t5052+t5056-t5400-t5689+t6300-t6493+t6497-t6540+t6541+t7004+t7615+t3385.*(t3417-t3421-t4507+t4513+t4519-t4540)+t6595.*(t3505.*1.838876e-2-t3570+t3571+t22.*(t1861-t3214).*(3.0./5.0e+2)+t22.*t23.*(t1861-t3214).*9.99471e-3);
et622 = t2388.*(-t3064+t4027+t3229.*(t1861-t3214).*9.840000000000001e-6)+t5426.*t6184+t5437.*t6185-t5798.*t6002-t5800.*t6005+t3057.*(-t3080+t4062+t17.*t3229.*(t1861-t3214).*1.02e-6);
et623 = -t5034-t5052+t5056-t5400-t5689+t6300-t6493+t6497-t6540+t6541+t7004+t7615+t3385.*(t3417-t3421-t4507+t4513+t4519-t4540)+t6595.*(t3505.*1.838876e-2-t3570+t3571+t22.*(t1861-t3214).*(3.0./5.0e+2)+t22.*t23.*(t1861-t3214).*9.99471e-3);
et624 = t2388.*(-t3064+t4027+t3229.*(t1861-t3214).*9.840000000000001e-6)+t5429.*t6184-t5799.*t6002-t5801.*t6005+t3057.*(-t3080+t4062+t17.*t3229.*(t1861-t3214).*1.02e-6)-t6185.*(t410-t5413);
et625 = (t6.*(et593+et594+et595+et596+et597))./2.0+(t7.*(t3047.*(-t5400+t6300-t6540+t6541+t3385.*(t3417-t3421-t4507+t4513+t4519-t4540)+t3057.*(-t3080+t4062+t17.*t3229.*(t1861-t3214).*1.02e-6))-t3957.*(t5357-t5512+t6671-t6674+t4541.*(t3417-t3421-t4507+t4513+t4519-t4540)+t6172.*(t3544-t4013))+t3946.*t7678-t17.*t2297.*t7318+t17.*t3483.*t7363+t17.*t7362.*(t1861-t3214)))./2.0+(t5.*(et607+et608+et609+et610+et611))./2.0-(t4.*(et617+et618+et619+et620))./2.0+(t2.*(et621+et622))./2.0;
et626 = (t3.*(et623+et624))./2.0;
et627 = t3563.*1.33637554986e-4+t3693-t3694+t33.*(t1896-t3232).*4.36041e-5;
et628 = t33.*t34.*(t1896-t3232).*7.26350557185e-5;
et629 = -t5204+t5522+t5705+t5775-t5782+t5892+t6234-t6240+t6450+t6949+t3877.*(t3959+t4200-t4287+t4409+t3996.*(t2801-t2850)+t3992.*(t335-t1539-t2831+t2851))+t6807.*(t2674-t2676+t3022-t3027)+(t2674-t2676+t3022-t3027).*(et627+et628).*(t1488+t1874+t2519+t2740+t2747+t3096+t3097)+t3617.*t4324.*(t2674-t2676+t3022-t3027)+t3689.*t5588.*(t2674-t2676+t3022-t3027)+t3313.*t3877.*(-t321+t332+t1196+t1212+t1237+t1238+t2139+t2140+t2159+t2165+t2754+t2814+t2953+t3072+t3405+t3412);
et630 = t3877.*t4134.*(t3410-t3708+t3714+t26.*t50.*t202.*(t46-t47).*8.687615694748404e-39)+t3877.*t5314.*(t1488+t1874+t2519+t2740+t2747+t3096+t3097);
et631 = t3563.*1.33637554986e-4+t3693-t3694+t33.*(t1896-t3232).*4.36041e-5;
et632 = t33.*t34.*(t1896-t3232).*7.26350557185e-5;
et633 = t3563.*1.33637554986e-4+t3693-t3694+t33.*(t1896-t3232).*4.36041e-5;
et634 = t33.*t34.*(t1896-t3232).*7.26350557185e-5;
et635 = (t4.*(et629+et630))./2.0-(t2.*t7868)./2.0+(t6.*t7995)./2.0-(t3.*(t3560+t3790+t3791+t3861+t3862+t4154+t4898-t5534-t5538+t5659+t5662-t5845-t5851+t5946+t5948+t6018+t6379+t6423+t6425+t5799.*(et631+et632)))./2.0+(t7.*(-t5515-t6054+t6147+t6956+t6961+t17.*t3483.*(t4311-t5186+t4541.*(-t2804+t2838+t3109+t23.*(t1456-t2355).*9.3e-7))))./2.0;
et636 = (t5.*(-t4963-t5685-t5687+t5785-t6028-t6317+t6321+t6600+t6608+t6863-t6864+t6869-t6871+t6994+t3210.*(t3959+t4200-t4287+t4409+t3996.*(t2801-t2850)+t3992.*(t335-t1539-t2831+t2851))+t3209.*(-t4196+t4285+t4582+t3206.*(t1896-t3232)+t3985.*(t2801-t2850)+t27.*t3863.*(t1896-t3232))+t6561.*(et633+et634)))./2.0;
et637 = t6023-t6048+t6210-t6625-t6656+t6657+t7057+t7066-t7223+t7224+t7302+t6986.*(t1477-t2502)+t3057.*(t3130+t3131+t3170+t3435-t4238-t4239-t4257+t4259-t4264+t4266-t4520-t4531+t4560+t4576+t2388.*(t1456-t2355).*4.0e-8+(t3524.*(t1861-t3214))./1.0e+8+(t3481.*(t1896-t3232))./1.0e+8-t17.*t2297.*t2363.*2.4e-7);
et638 = t2363.*(t3156+t3157+t3376-t4255-t4256-t4499+t4504+t3524.*(t1861-t3214).*6.2e-7+t3481.*(t1896-t3232).*6.2e-7-(t17.*(t1861-t3214).*(t1896-t3232))./1.0e+8-(t17.*t2297.*t2363)./1.0e+8-(t17.*t3483.*t3528)./1.0e+8)+t5800.*(t4874+t5148-t5704-t6318);
et639 = t27.*t2363.*(-t3423+t4543+t3946.*(t1896-t3232).*1.02e-6);
et640 = t6023-t6048+t6210-t6625-t6656+t6657+t7057+t7066-t7223+t7224+t7304+t6986.*(t1477-t2502)+t3057.*(t3130+t3131+t3170+t3435-t4238-t4239-t4257+t4259-t4264+t4266-t4520-t4531+t4560+t4576+t2388.*(t1456-t2355).*4.0e-8+(t3524.*(t1861-t3214))./1.0e+8+(t3481.*(t1896-t3232))./1.0e+8-t17.*t2297.*t2363.*2.4e-7);
et641 = t2363.*(t3156+t3157+t3376-t4255-t4256-t4499+t4504+t3524.*(t1861-t3214).*6.2e-7+t3481.*(t1896-t3232).*6.2e-7-(t17.*(t1861-t3214).*(t1896-t3232))./1.0e+8-(t17.*t2297.*t2363)./1.0e+8-(t17.*t3483.*t3528)./1.0e+8)+t5801.*(t4874+t5148-t5704-t6318);
et642 = t27.*t2363.*(-t3423+t4543+t3946.*(t1896-t3232).*1.02e-6);
et643 = t2.*t7993+t3.*t7994+(t7.*t8025)./2.0+t6.*t8027-t5.*t8033-(t4.*t8038)./2.0-(t5.*t8044)./2.0+(t6.*t8047)./2.0+t7.*(t7391+t7395-t7702+t3957.*(t5654+t5655-t6370-t6638-t6641+t6039.*(t3544-t4013))+t7318.*(t1456-t2355)+t3047.*(t5436+t5438+t6119+t6122+t6536+t6538))-t4.*(-t4496+t4650-t5227+t5443-t5890+t6101+t6485+t6894+t7611+t7613+t7698+t7676.*(t2674-t2676+t3022-t3027)+t4134.*t5486.*(t2674-t2676+t3022-t3027)+t3782.*t6183.*(t2674-t2676+t3022-t3027)+t3892.*t6595.*(t2674-t2676+t3022-t3027)+t3877.*t5738.*(t1488+t1874+t2519+t2740+t2747+t3096+t3097))-(t2.*(et637+et638+et639))./2.0;
et644 = t3.*(et640+et641+et642).*(-1.0./2.0);
et645 = t3563.*1.33637554986e-4+t3693-t3694+t33.*(t1896-t3232).*4.36041e-5;
et646 = t33.*t34.*(t1896-t3232).*7.26350557185e-5;
et647 = -t5204+t5522+t5707+t5711+t5775-t5782+t5894+t6237-t6242+t6450+t6949+t3877.*(t3959+t4200-t4287+t4409+t3996.*(t2801-t2850)+t3992.*(t335-t1539-t2831+t2851))+t6807.*(t2674-t2676+t3022-t3027)+(t2674-t2676+t3022-t3027).*(et645+et646).*(t1488+t1874+t2519+t2740+t2747+t3096+t3097)+t3617.*t4324.*(t2674-t2676+t3022-t3027)+t3689.*t5589.*(t2674-t2676+t3022-t3027);
et648 = t3877.*t4134.*(t3410-t3708+t3714+t26.*t50.*t202.*(t46-t47).*8.687615694748404e-39)+t3877.*t5314.*(t1488+t1874+t2519+t2740+t2747+t3096+t3097);
et649 = t3563.*1.33637554986e-4+t3693-t3694+t33.*(t1896-t3232).*4.36041e-5;
et650 = t33.*t34.*(t1896-t3232).*7.26350557185e-5;
et651 = t1288+t1289+t1302+t1303-t1319-t1320+t1336-t1348+t1350+t1351-t1360+t1369-t1378+t1396-t1425+t1435-t2174+t2183-t2187+t2193-t2194-t2195+t2199-t2203-t2215+t2219-t2222-t2223+t2239+t2240-t2256-t2257+t2555+t2556+t2572+t2583-t2605-t2606+t2612+t2613-t2618-t2619+t2651+t2652;
et652 = t24.*t25.*t26.*t50.*t202.*(-3.566935413776081e-21);
et653 = t30.*t31.*t32.*t50.*t202.*(-3.992732227073824e-24);
et654 = t24.*t25.*t32.*t33.*t50.*t202.*(-3.509445006623964e-21);
et655 = t27.*t30.*t31.*t32.*t50.*t202.*(-7.696420262413979e-21);
et656 = (t2.*t7870)./2.0+(t3.*t7872)./2.0+(t6.*t7996)./2.0+(t4.*(et647+et648))./2.0+(t7.*(-t5515-t6054+t6147+t6956+t6961+t17.*t3483.*(t4311-t5186+t4541.*(-t2804+t2838+t3109+t23.*(t1456-t2355).*9.3e-7))))./2.0;
et657 = (t5.*(-t4963-t5685-t5687+t5785-t6028-t6317+t6321+t6604+t6611+t6863-t6866+t6869-t6872+t6994+t3210.*(t3959+t4200-t4287+t4409+t3996.*(t2801-t2850)+t3992.*(t335-t1539-t2831+t2851))+t3209.*(-t4196+t4285+t4582+t3206.*(t1896-t3232)+t3985.*(t2801-t2850)+t27.*t3863.*(t1896-t3232))+t6561.*(et649+et650)))./2.0+t2.*(t6753+t6763-t6765+t7138-t7140-t7142+t7145+t5412.*(et651+et652+et653+et654+et655));
et658 = -t2306-t2317+t3144+t3147+t35.*t941.*t948.*(t850-t874).*3.775747223193135e-1;
et659 = t36.*t941.*t948.*(t850-t874).*2.244797987218524e-1;
et660 = -t2306-t2317+t3144+t3147+t35.*t941.*t948.*(t850-t874).*3.775747223193135e-1;
et661 = t36.*t941.*t948.*(t850-t874).*2.244797987218524e-1;
et662 = -t2306-t2317+t3144+t3147+t35.*t941.*t948.*(t850-t874).*3.775747223193135e-1;
et663 = t36.*t941.*t948.*(t850-t874).*2.244797987218524e-1;
et664 = t4219+t4242+t4663+t4702-t5245-t5246-t5247-t5248+t5345+t5348-t5433-t5434-t5440-t5441+t7295-t7297+t7776-t7782+t3877.*(t5582+t5715-t6598-t6801+t6802+t6413.*(t3544-t4013))+t7757.*(t2674-t2676+t3022-t3027)+t3984.*(t2674-t2676+t3022-t3027).*(t2694-t2701+t3036-t3043).*(t1488+t1874+t2519+t2740+t2747+t3096+t3097).*7.26735e-3;
et665 = t3941.*(t2674-t2676+t3022-t3027).*(t2694-t2701+t3036-t3043).*(t1513+t1879+t2598+t2820+t2834+t3117+t3118).*7.26735e-3+t3877.*t3901.*t3984.*(t1488+t1874+t2519+t2740+t2747+t3096+t3097).*7.26735e-3+t3877.*t3901.*t3941.*(t1513+t1879+t2598+t2820+t2834+t3117+t3118).*7.26735e-3;
et666 = -t5196-t5322-t5330+t5331+t5335+t5504+t5506+t5558+t5810-t5969+t6113-t6117+t7693+t7735+(t2694-t2701+t3036-t3043).*(t3505.*1.838876e-2-t3570+t3571+t22.*(t1861-t3214).*(3.0./5.0e+2)+t22.*t23.*(t1861-t3214).*9.99471e-3).*(t1513+t1879+t2598+t2820+t2834+t3117+t3118).*7.26735e-3;
et667 = t3628.*t4277.*(t2694-t2701+t3036-t3043).*2.889644e-2+t3732.*t5426.*(t2694-t2701+t3036-t3043).*1.08769e-2+t3359.*t3901.*(-t56+t60+t649+t670+t686+t687+t1577+t1578+t1586+t1600+t2303+t2339+t2689+t3030+t3292+t3305).*2.889644e-2;
et668 = t3901.*t5220.*(t1513+t1879+t2598+t2820+t2834+t3117+t3118).*7.26735e-3;
et669 = t1288+t1289+t1302+t1303-t1319-t1320+t1336-t1348+t1350+t1351-t1360+t1369-t1378+t1396-t1425+t1435-t2174+t2183-t2187+t2193-t2194-t2195+t2199-t2203-t2215+t2219-t2222-t2223+t2239+t2240-t2256-t2257+t2555+t2556+t2572+t2583-t2605-t2606+t2612+t2613-t2618-t2619+t2651+t2652;
et670 = t24.*t25.*t26.*t50.*t202.*(-3.566935413776081e-21);
et671 = t30.*t31.*t32.*t50.*t202.*(-3.992732227073824e-24);
et672 = t24.*t25.*t32.*t33.*t50.*t202.*(-3.509445006623964e-21);
et673 = t27.*t30.*t31.*t32.*t50.*t202.*(-7.696420262413979e-21);
et674 = t4.*(-t4911+t5005-t5488+t5578-t6206+t6207+t6508+t6689-t6692+t6940+t7086+t7359+t7424+t7444+t7446-t7733-t7734-t7897-t7898+t7917-t7919+t6975.*(et658+et659)+t7326.*(et660+et661)+t7363.*(et662+et663)+t4822.*(-t5209+t5751+t5639.*(t1896-t3232))+t3891.*t6183.*(t2674-t2676+t3022-t3027)+t4298.*t6595.*(t2674-t2676+t3022-t3027)+t4822.*t6595.*(t1488+t1874+t2519+t2740+t2747+t3096+t3097))-(t4.*(et664+et665))./2.0-(t2.*(et666+et667+et668))./2.0;
et675 = t5.*(t4868+t4869-t5620+t5626+t6809-t6811+t6812-t6892+t7054+t7299+t7319-t7336-t7389+t7579+t7581+t7583-t7665-t7730+t7731+t7854+t7865+t7892-t7894-t7910-t7911+t5723.*(et669+et670+et671+et672+et673)+t6564.*(t4983-t5225-t6233+t7058)+t6975.*(-t1901+t3122+t3270)+t7326.*(-t1901+t3122+t3270)+t7363.*(-t1901+t3122+t3270))+t2.*t8035+t3.*t8036+(t5.*t8040)./2.0-(t6.*t8045)./2.0+t6.*t8049+t7.*(t7322-t7422+t7871-t7920-t7921+t7363.*(t17.*((t237.*(t42-t43))./9.007199254740992e+15+t21.*(-t1881+t3121+t3269))+t22.*(-t1901+t3122+t3270)));
et676 = t7.*(-t7356+t7466+t7700-t7779+t3957.*(t5582+t5715-t6598-t6801+t6802+t6413.*(t3544-t4013))+t17.*t7440.*(t1861-t3214)).*(-1.0./2.0)+(t3.*(t5196+t5322+t5330-t5331-t5335-t5365+t5505+t5507+t5561+t5575+t5585+t5809+t5813+t5832+t5833+t5969+t5997+t6020+t6116+t6118+t6124+t6348+t6477+t6478+t6534+t6697+t6698+t6777-t3628.*t4277.*(t2694-t2701+t3036-t3043).*2.889644e-2))./2.0;
et677 = (t2.*(t5762-t6289-t6936+t6938+t7266-t7268))./2.0+(t3.*(t5762-t6289-t6936+t6938+t7266-t7268))./2.0+(t6.*(-t7494+t7541-t7545+t7851+t2297.*(t5762-t6289-t6936+t6938+t7266-t7268)+t7846.*(t1861-t3214)))./2.0+t7.*t7978+t4.*t7983-(t4.*t7997)./2.0+t5.*t8003-t6.*t8004-(t5.*t8015)./2.0-(t7.*t8031)./2.0;
et678 = t2.*(-t6613-t6615+t7047+t7616+t6595.*(-t4007+t4011+t18.*(t1861-t3214).*1.838876e-2+t23.*(t1861-t3214).*9.99471e-3));
et679 = t3.*(-t6614-t6616+t7047+t7616+t6595.*(-t4007+t4011+t18.*(t1861-t3214).*1.838876e-2+t23.*(t1861-t3214).*9.99471e-3));
et680 = t6030-t6943-t6945+t3942.*(t4510.*(t2813-t2835+t18.*(t1456-t2355).*1.02e-6+t23.*(t1456-t2355).*9.0e-8)+t4514.*(-t2804+t2838+t3109+t23.*(t1456-t2355).*9.3e-7)+t3132.*(t3235-t3535))+t5489.*(t1456-t2355);
et681 = t3967.*(t4311-t5186+t4541.*(-t2804+t2838+t3109+t23.*(t1456-t2355).*9.3e-7));
et682 = t707+t708-t721-t722-t749+t762+t768-t777-t792-t793-t801-t802-t808+t813-t819+t821-t1629+t1637-t1640-t1641-t1659-t1661+t1666+t1667+t1683+t1692+t1705-t1712+t1758+t1759+t1775+t1776+t1973+t1993+t1994+t2023+t2053+t2060-t2089-t2090+t2098+t2099-t14.*t15.*t21.*t50.*t189.*3.670836568391568e-22;
et683 = t16.*t19.*t20.*t50.*t189.*(-3.279367663374749e-19)-t14.*t15.*t17.*t21.*t50.*t189.*7.075931802640439e-19;
et684 = t14.*t17.*t20.*t21.*t50.*t189.*(-1.190170786299927e-18)-t15.*t17.*t19.*t21.*t50.*t189.*1.190170786299927e-18;
et685 = t19.*t20.*t21.*t22.*t50.*t189.*(-3.226512155691387e-19);
et686 = -t5760+t6009+t6104-t6356+t6387-t6392+t6623+t6628-t6854-t6857+t7006+t5223.*(t350+t366-t1205+t1210-t1217-t1218-t2147+t2152+t2154+t2155-t3395-t3399-t3409-t3716+t3723+t32.*t50.*t202.*(t46-t47).*8.687615694748404e-39)+t4975.*(et682+et683+et684+et685);
et687 = t6561.*(t3349-t3649+t28.*(t3235-t3535).*1.33637554986e-4+t34.*(t3235-t3535).*7.26350557185e-5);
et688 = t5031-t7091+t4795.*(t1005+t26.*(t1941-t3308+t39.*t1022.*(t855-t878).*2.196325630278387e-1)).*7.26735e-3;
et689 = t2419.*(t684+t685-t710+t724+t1686-t1690+t1700+t1701+t2371+t2698+t2707-t2716+t2719+t3319-t3327-t3341-t3620+t3622+t3634-t3638+t4076+t4077).*7.26735e-3;
et690 = -t5518-t5531+t7331+t7342-t7405+t7448+t7450+t7587-t7598+t7900+t7904+t7922-t7935+t7936+t6561.*(et688+et689)+t7353.*(t4795.*(t1896-t3232).*7.26735e-3+t2363.*(t684+t685-t710+t724+t1686-t1690+t1700+t1701+t2371+t2698+t2707-t2716+t2719+t3319-t3327-t3341-t3620+t3622+t3634-t3638+t4076+t4077).*7.26735e-3);
et691 = t3882.*(t6767+t6001.*(t1896-t3232)+t3985.*(t3424-t3437+t4552+t4556+t3942.*(t1896-t3232).*5.7e-7+t3946.*(t1896-t3232).*4.0e-8));
et692 = t3210.*(t6179-t6903-t7211+t7282+t7453+t4824.*(t3424-t3437+t4552+t4556+t3942.*(t1896-t3232).*5.7e-7+t3946.*(t1896-t3232).*4.0e-8));
et693 = t5592+t5594+t5822+t5836+t6108+t6389-t6391-t6675-t6676+t7621+t3057.*(t4752+t3942.*(t2694-t2701+t3036-t3043).*1.02e-6)+t5520.*(t1477-t2502)+t3784.*t5426.*(t2694-t2701+t3036-t3043).*1.08769e-2+t3918.*t5798.*(t2694-t2701+t3036-t3043).*7.26735e-3;
et694 = t3901.*t5262.*(t1513+t1879+t2598+t2820+t2834+t3117+t3118).*7.26735e-3;
et695 = t5592+t5594+t5824+t5836+t6110+t6389-t6391-t6675-t6676+t7621+t3057.*(t4752+t3942.*(t2694-t2701+t3036-t3043).*1.02e-6)+t5520.*(t1477-t2502)+t3784.*t5429.*(t2694-t2701+t3036-t3043).*1.08769e-2+t3918.*t5799.*(t2694-t2701+t3036-t3043).*7.26735e-3;
et696 = t3901.*t5262.*(t1513+t1879+t2598+t2820+t2834+t3117+t3118).*7.26735e-3;
et697 = -t2306-t2317+t3144+t3147+t35.*t941.*t948.*(t850-t874).*3.775747223193135e-1;
et698 = t36.*t941.*t948.*(t850-t874).*2.244797987218524e-1;
et699 = t707+t708-t721-t722-t749+t762+t768-t777-t792-t793-t801-t802-t808+t813-t819+t821-t1629+t1637-t1640-t1641-t1659-t1661+t1666+t1667+t1683+t1692+t1705-t1712+t1758+t1759+t1775+t1776+t1973+t1993+t1994+t2023+t2053+t2060-t2089-t2090+t2098+t2099-t14.*t15.*t21.*t50.*t189.*3.670836568391568e-22;
et700 = t16.*t19.*t20.*t50.*t189.*(-3.279367663374749e-19)-t14.*t15.*t17.*t21.*t50.*t189.*7.075931802640439e-19;
et701 = t14.*t17.*t20.*t21.*t50.*t189.*(-1.190170786299927e-18)-t15.*t17.*t19.*t21.*t50.*t189.*1.190170786299927e-18;
et702 = t19.*t20.*t21.*t22.*t50.*t189.*(-3.226512155691387e-19);
et703 = -t4615+t4640-t5252+t5427-t5791+t6089+t6851+t7652+t7655+t7683+t7755+t3209.*(-t5772-t5773+t6522+t6523+t28.*t6620.*(t3235-t3535)+t34.*t6617.*(t3235-t3535))+t4175.*t5224.*(t2694-t2701+t3036-t3043).*1.08769e-2+t3784.*t5951.*(t2694-t2701+t3036-t3043).*1.08769e-2;
et704 = t3918.*t6561.*(t2694-t2701+t3036-t3043).*7.26735e-3+t3784.*t3901.*(et699+et700+et701+et702).*1.08769e-2+t3901.*t5713.*(t1513+t1879+t2598+t2820+t2834+t3117+t3118).*7.26735e-3+t50.*t189.*(t5563+t6360+t6361+t6362+t6795).*9.543032792050485e-17;
et705 = (t4.*t8012)./2.0+t2.*t8023+t3.*t8024-(t6.*t8029)./2.0+t6.*t8051+t5.*(et690+et691+et692)-(t2.*(et693+et694))./2.0-(t3.*(et695+et696))./2.0;
et706 = -t4.*(t5388+t5491-t6984-t6985-t7099-t7100+t7432+t7478+t7488+t7927+t7929-t7943+t4822.*(t6767+t6001.*(t1896-t3232)+t3985.*(t3424-t3437+t4552+t4556+t3942.*(t1896-t3232).*5.7e-7+t3946.*(t1896-t3232).*4.0e-8))+t7933.*(t2674-t2676+t3022-t3027)+t7417.*(et697+et698)+t3877.*t7398.*(t1488+t1874+t2519+t2740+t2747+t3096+t3097))+(t5.*(et703+et704))./2.0;
et707 = t7.*(t7474+t7476+t7771-t7773+t7352.*(t1456-t2355)+t3047.*(t6389-t6391-t6675-t6676+t3057.*(t4752+t3942.*(t2694-t2701+t3036-t3043).*1.02e-6)+t5520.*(t1477-t2502))).*(-1.0./2.0)+t7.*(t7486+t7487+t7907+t7947+t7948-t2994.*(-t6677+t6681+t3057.*(-t3423+t4543+t3946.*(t1896-t3232).*1.02e-6)));
et708 = t6023-t6048+t6210-t6625-t6656+t6657+t7057+t7066-t7223+t7224+t7302+t6986.*(t1477-t2502)+t3057.*(t3130+t3131+t3170+t3435-t4238-t4239-t4257+t4259-t4264+t4266-t4520-t4531+t4560+t4576+t2388.*(t1456-t2355).*4.0e-8+(t3524.*(t1861-t3214))./1.0e+8+(t3481.*(t1896-t3232))./1.0e+8-t17.*t2297.*t2363.*2.4e-7);
et709 = t2363.*(t3156+t3157+t3376-t4255-t4256-t4499+t4504+t3524.*(t1861-t3214).*6.2e-7+t3481.*(t1896-t3232).*6.2e-7-(t17.*(t1861-t3214).*(t1896-t3232))./1.0e+8-(t17.*t2297.*t2363)./1.0e+8-(t17.*t3483.*t3528)./1.0e+8)+t5800.*(t4874+t5148-t5704-t6318);
et710 = t27.*t2363.*(-t3423+t4543+t3946.*(t1896-t3232).*1.02e-6);
et711 = t6023-t6048+t6210-t6625-t6656+t6657+t7057+t7066-t7223+t7224+t7304+t6986.*(t1477-t2502)+t3057.*(t3130+t3131+t3170+t3435-t4238-t4239-t4257+t4259-t4264+t4266-t4520-t4531+t4560+t4576+t2388.*(t1456-t2355).*4.0e-8+(t3524.*(t1861-t3214))./1.0e+8+(t3481.*(t1896-t3232))./1.0e+8-t17.*t2297.*t2363.*2.4e-7);
et712 = t2363.*(t3156+t3157+t3376-t4255-t4256-t4499+t4504+t3524.*(t1861-t3214).*6.2e-7+t3481.*(t1896-t3232).*6.2e-7-(t17.*(t1861-t3214).*(t1896-t3232))./1.0e+8-(t17.*t2297.*t2363)./1.0e+8-(t17.*t3483.*t3528)./1.0e+8)+t5801.*(t4874+t5148-t5704-t6318);
et713 = t27.*t2363.*(-t3423+t4543+t3946.*(t1896-t3232).*1.02e-6);
et714 = (t2.*t7993)./2.0+(t3.*t7994)./2.0+t7.*t8025+(t6.*t8027)./2.0-(t5.*t8033)./2.0-t4.*t8038-t5.*t8044+t6.*t8047+(t7.*(t7391+t7395-t7702+t3957.*(t5654+t5655-t6370-t6638-t6641+t6039.*(t3544-t4013))+t7318.*(t1456-t2355)+t3047.*(t5436+t5438+t6119+t6122+t6536+t6538)))./2.0-(t4.*(-t4496+t4650-t5227+t5443-t5890+t6101+t6485+t6894+t7611+t7613+t7698+t7676.*(t2674-t2676+t3022-t3027)+t4134.*t5486.*(t2674-t2676+t3022-t3027)+t3782.*t6183.*(t2674-t2676+t3022-t3027)+t3892.*t6595.*(t2674-t2676+t3022-t3027)+t3877.*t5738.*(t1488+t1874+t2519+t2740+t2747+t3096+t3097)))./2.0-t2.*(et708+et709+et710);
et715 = -t3.*(et711+et712+et713);
et716 = t3681+t3684-t3834+t4849+t4857-t5104+t5105-t5136+t3360.*(t1477-t2502).*9.3e-7+t3996.*(t3493-t3972).*9.0e-8+t18.*t3946.*(t3235-t3535).*9.0e-8;
et717 = t23.*t3946.*(t3235-t3535).*9.3e-7;
et718 = t3209;
et719 = -t5877-t6660+t4514.*(et716+et717)+t4510.*(t3680+t3685-t3827+t4848+t4856-t5103+t5111-t5140+t18.*t4833+t3360.*(t1477-t2502).*9.0e-8+t3996.*(t3493-t3972).*1.02e-6+t23.*t3946.*(t3235-t3535).*9.0e-8)+t28.*t6899.*(t3235-t3535)+t34.*t6898.*(t3235-t3535);
et720 = (t2.*(t6929+t6930+t7288+t7290-t5739.*(t1477-t2502)-t3057.*(t4819+t4850+t4851+t3057.*(t1456-t2355).*1.02e-6+t3047.*(t1477-t2502).*1.02e-6+t3942.*(t3235-t3535).*1.02e-6)))./2.0;
et721 = (t3.*(t6929+t6930+t7288+t7290-t5739.*(t1477-t2502)-t3057.*(t4819+t4850+t4851+t3057.*(t1456-t2355).*1.02e-6+t3047.*(t1477-t2502).*1.02e-6+t3942.*(t3235-t3535).*1.02e-6)))./2.0+t2.*t7888+t3.*t7889+t7.*t7984+(t4.*t8000)./2.0+t5.*t8005-t6.*t8006+(t6.*t8018)./2.0;
et722 = t7.*t8034.*(-1.0./2.0)+t4.*(t5240-t5384-t6236+t6972+t6976+t7712+t7690.*(t2674-t2676+t3022-t3027)+(t4610+t2363.*(t3547.*1.838876e-2+t4071-t4072+t34.*(t1896-t3232).*9.99471e-3).*7.26735e-3).*(t2674-t2676+t3022-t3027).*(t1488+t1874+t2519+t2740+t2747+t3096+t3097))+(t5.*(t7841-t7877+et718.*et719))./2.0;
et723 = t5621+t5628+t5919+t6226-t6453-t6459+t6932-t6934+t3782.*t5588.*(t2674-t2676+t3022-t3027)+t3892.*t5884.*(t2674-t2676+t3022-t3027);
et724 = (t3349-t3649+t28.*(t3235-t3535).*1.33637554986e-4+t34.*(t3235-t3535).*7.26350557185e-5).*(t2674-t2676+t3022-t3027).*(t1488+t1874+t2519+t2740+t2747+t3096+t3097)+t3877.*t5321.*(t1488+t1874+t2519+t2740+t2747+t3096+t3097);
et725 = t5740+t5743+t4514.*(t4555+t4571-t18.*t2363.*t3047.*9.0e-8-t23.*t2363.*t3047.*9.3e-7+t18.*t3946.*(t1896-t3232).*9.0e-8+t23.*t3946.*(t1896-t3232).*9.3e-7);
et726 = t4510.*(t4554+t4572-t18.*t2363.*t3047.*1.02e-6-t23.*t2363.*t3047.*9.0e-8+t18.*t3946.*(t1896-t3232).*1.02e-6+t23.*t3946.*(t1896-t3232).*9.0e-8);
et727 = t28.*t6588.*(t3235-t3535)+t34.*t6587.*(t3235-t3535);
et728 = t6561.*(t4323.*(t1896-t3232).*7.26735e-3+t2363.*(t3318+t3334+t3621-t3637+t28.*(t3235-t3535).*1.838876e-2+t34.*(t3235-t3535).*9.99471e-3).*7.26735e-3);
et729 = -t5710.*(t4795.*(t1896-t3232).*7.26735e-3+t2363.*(t684+t685-t710+t724+t1686-t1690+t1700+t1701+t2371+t2698+t2707-t2716+t2719+t3319-t3327-t3341-t3620+t3622+t3634-t3638+t4076+t4077).*7.26735e-3)+t3209.*t7624-t3210.*t7740-t5713.*t6696+t6007.*t6564;
et730 = t3210.*(t5612-t6399-t6401+t6770+t3992.*(t3424-t3437+t4552+t4556+t3942.*(t1896-t3232).*5.7e-7+t3946.*(t1896-t3232).*4.0e-8))+t3209.*(et725+et726+et727)-t50.*t189.*(t5527+t5528+t6303+t6304+t6647+t6648).*9.543032792050485e-17;
et731 = t50.*t189.*t7602.*(-9.543032792050485e-17);
et732 = t236.*t241.*t3940.*t4792.*(-2.595777943136013e-110);
et733 = t236.*t241.*t4789.*t4974.*2.595777943136013e-110;
et734 = t4323.*(t1896-t3232).*7.26735e-3+t2363.*(t3318+t3334+t3621-t3637+t28.*(t3235-t3535).*1.838876e-2+t34.*(t3235-t3535).*9.99471e-3).*7.26735e-3;
et735 = -(t4758.*(t1861-t3214)+t2297.*(t642+t643-t667+t674+t1587+t1606+t1608+t1609+t2295+t2671+t2683+t2684-t2695+t3272+t3290-t3296+t3576+t3582+t3588-t3593+t4015+t4016));
et736 = t5740+t5743+t4514.*(t4555+t4571-t18.*t2363.*t3047.*9.0e-8-t23.*t2363.*t3047.*9.3e-7+t18.*t3946.*(t1896-t3232).*9.0e-8+t23.*t3946.*(t1896-t3232).*9.3e-7);
et737 = t4510.*(t4554+t4572-t18.*t2363.*t3047.*1.02e-6-t23.*t2363.*t3047.*9.0e-8+t18.*t3946.*(t1896-t3232).*1.02e-6+t23.*t3946.*(t1896-t3232).*9.0e-8);
et738 = t28.*t6588.*(t3235-t3535)+t34.*t6587.*(t3235-t3535);
et739 = -t5983.*(t4795.*(t1896-t3232).*7.26735e-3+t2363.*(t684+t685-t710+t724+t1686-t1690+t1700+t1701+t2371+t2698+t2707-t2716+t2719+t3319-t3327-t3341-t3620+t3622+t3634-t3638+t4076+t4077).*7.26735e-3)+t2297.*t7602-t3483.*t7740-t6007.*t6631-t5985.*t6696+et734.*et735;
et740 = t3483.*(t5612-t6399-t6401+t6770+t3992.*(t3424-t3437+t4552+t4556+t3942.*(t1896-t3232).*5.7e-7+t3946.*(t1896-t3232).*4.0e-8))+t7624.*(t1861-t3214)+(t1861-t3214).*(et736+et737+et738)+t2297.*(t5527+t5528+t6303+t6304+t6647+t6648);
et741 = t236.*t241.*t4705.*t4789.*5.316153227542554e-107;
et742 = t236.*t241.*t4704.*t4792.*5.316153227542554e-107;
et743 = t5740+t5743+t4514.*(t4555+t4571-t18.*t2363.*t3047.*9.0e-8-t23.*t2363.*t3047.*9.3e-7+t18.*t3946.*(t1896-t3232).*9.0e-8+t23.*t3946.*(t1896-t3232).*9.3e-7);
et744 = t4510.*(t4554+t4572-t18.*t2363.*t3047.*1.02e-6-t23.*t2363.*t3047.*9.0e-8+t18.*t3946.*(t1896-t3232).*1.02e-6+t23.*t3946.*(t1896-t3232).*9.0e-8);
et745 = t28.*t6588.*(t3235-t3535)+t34.*t6587.*(t3235-t3535);
et746 = -t3877.*t7740+t3877.*(t5612-t6399-t6401+t6770+t3992.*(t3424-t3437+t4552+t4556+t3942.*(t1896-t3232).*5.7e-7+t3946.*(t1896-t3232).*4.0e-8))+t7624.*(t2674-t2676+t3022-t3027)+(t2674-t2676+t3022-t3027).*(et743+et744+et745);
et747 = -t3892.*(t4795.*(t1896-t3232).*7.26735e-3+t2363.*(t684+t685-t710+t724+t1686-t1690+t1700+t1701+t2371+t2698+t2707-t2716+t2719+t3319-t3327-t3341-t3620+t3622+t3634-t3638+t4076+t4077).*7.26735e-3).*(t2674-t2676+t3022-t3027);
et748 = (t4323.*(t1896-t3232).*7.26735e-3+t2363.*(t3318+t3334+t3621-t3637+t28.*(t3235-t3535).*1.838876e-2+t34.*(t3235-t3535).*9.99471e-3).*7.26735e-3).*(t2674-t2676+t3022-t3027).*(t1488+t1874+t2519+t2740+t2747+t3096+t3097);
et749 = -t3877.*t3892.*t6696+t3877.*t6007.*(t1488+t1874+t2519+t2740+t2747+t3096+t3097)+t236.*t241.*t4220.*t4792.*4.788365138921021e-91;
et750 = t236.*t241.*t4644.*t4789.*4.788365138921021e-91;
et751 = t5740+t5743+t4514.*(t4555+t4571-t18.*t2363.*t3047.*9.0e-8-t23.*t2363.*t3047.*9.3e-7+t18.*t3946.*(t1896-t3232).*9.0e-8+t23.*t3946.*(t1896-t3232).*9.3e-7);
et752 = t4510.*(t4554+t4572-t18.*t2363.*t3047.*1.02e-6-t23.*t2363.*t3047.*9.0e-8+t18.*t3946.*(t1896-t3232).*1.02e-6+t23.*t3946.*(t1896-t3232).*9.0e-8);
et753 = t28.*t6588.*(t3235-t3535)+t34.*t6587.*(t3235-t3535);
et754 = t5.*(et728+et729+et730+et731+et732+et733).*(-1.0./2.0)+(t6.*(et739+et740+et741+et742))./2.0-(t4.*(et746+et747+et748+et749+et750))./2.0;
et755 = (t2.*(t5527+t5528+t6303+t6304+t6647+t6648+t7068+t7070+t7602+t5798.*(t4323.*(t1896-t3232).*7.26735e-3+t2363.*(t3318+t3334+t3621-t3637+t28.*(t3235-t3535).*1.838876e-2+t34.*(t3235-t3535).*9.99471e-3).*7.26735e-3)+t5800.*t6007))./2.0;
et756 = (t3.*(t5527+t5528+t6303+t6304+t6647+t6648+t7068+t7070+t7602+t5799.*(t4323.*(t1896-t3232).*7.26735e-3+t2363.*(t3318+t3334+t3621-t3637+t28.*(t3235-t3535).*1.838876e-2+t34.*(t3235-t3535).*9.99471e-3).*7.26735e-3)+t5801.*t6007))./2.0;
et757 = (t7.*(t3942.*t7416+t3967.*t7417+t3957.*t7740-t3946.*(et751+et752+et753)+(t1456-t2355).*(-t6677+t6681+t3057.*(-t3423+t4543+t3946.*(t1896-t3232).*1.02e-6))+t3047.*(t5527+t5528+t6303+t6304+t6647+t6648)))./2.0;
et758 = t3681+t3684-t3834+t4849+t4857-t5104+t5105-t5136+t3360.*(t1477-t2502).*9.3e-7+t3996.*(t3493-t3972).*9.0e-8+t18.*t3946.*(t3235-t3535).*9.0e-8;
et759 = t23.*t3946.*(t3235-t3535).*9.3e-7;
et760 = t3209;
et761 = -t5877-t6660+t4514.*(et758+et759)+t4510.*(t3680+t3685-t3827+t4848+t4856-t5103+t5111-t5140+t18.*t4833+t3360.*(t1477-t2502).*9.0e-8+t3996.*(t3493-t3972).*1.02e-6+t23.*t3946.*(t3235-t3535).*9.0e-8)+t28.*t6899.*(t3235-t3535)+t34.*t6898.*(t3235-t3535);
et762 = t2.*(t6929+t6930+t7288+t7290-t5739.*(t1477-t2502)-t3057.*(t4819+t4850+t4851+t3057.*(t1456-t2355).*1.02e-6+t3047.*(t1477-t2502).*1.02e-6+t3942.*(t3235-t3535).*1.02e-6));
et763 = t3.*(t6929+t6930+t7288+t7290-t5739.*(t1477-t2502)-t3057.*(t4819+t4850+t4851+t3057.*(t1456-t2355).*1.02e-6+t3047.*(t1477-t2502).*1.02e-6+t3942.*(t3235-t3535).*1.02e-6))+(t2.*t7888)./2.0+(t3.*t7889)./2.0+(t7.*t7984)./2.0+t4.*t8000+(t5.*t8005)./2.0-(t6.*t8006)./2.0;
et764 = t6.*t8018-t7.*t8034+(t4.*(t5240-t5384-t6236+t6972+t6976+t7712+t7690.*(t2674-t2676+t3022-t3027)+(t4610+t2363.*(t3547.*1.838876e-2+t4071-t4072+t34.*(t1896-t3232).*9.99471e-3).*7.26735e-3).*(t2674-t2676+t3022-t3027).*(t1488+t1874+t2519+t2740+t2747+t3096+t3097)))./2.0+t5.*(t7841-t7877+et760.*et761);
et765 = (t7.*(t3047.*t7741-t3957.*t7784+t3946.*(t7072-t7077+t4514.*(t3817-t5119-t5134+t5135+t3057.*(t2337+t18.*(t1456-t2355)).*9.3e-7+t4491.*(t3235-t3535).*9.3e-7)+t4510.*(t3811+t3833-t5114+t5117-t5133+t5139))))./2.0;
et766 = (t5.*(-t3210.*t7784+t3209.*(t7072-t7077+t4514.*(t3817-t5119-t5134+t5135+t3057.*(t2337+t18.*(t1456-t2355)).*9.3e-7+t4491.*(t3235-t3535).*9.3e-7)+t4510.*(t3811+t3833-t5114+t5117-t5133+t5139))+t50.*t189.*t7741.*9.543032792050485e-17))./2.0;
et767 = t4.*(t3877.*t7784-(t7072-t7077+t4514.*(t3817-t5119-t5134+t5135+t3057.*(t2337+t18.*(t1456-t2355)).*9.3e-7+t4491.*(t3235-t3535).*9.3e-7)+t4510.*(t3811+t3833-t5114+t5117-t5133+t5139)).*(t2674-t2676+t3022-t3027)).*(-1.0./2.0);
et768 = (t6.*(t2297.*t7741+t3483.*t7784-(t1861-t3214).*(t7072-t7077+t4514.*(t3817-t5119-t5134+t5135+t3057.*(t2337+t18.*(t1456-t2355)).*9.3e-7+t4491.*(t3235-t3535).*9.3e-7)+t4510.*(t3811+t3833-t5114+t5117-t5133+t5139))))./2.0+(t2.*t7741)./2.0+(t3.*t7741)./2.0;
et769 = t2.*(t5762-t6289-t6936+t6938+t7266-t7268)+t3.*(t5762-t6289-t6936+t6938+t7266-t7268)+t6.*(-t7494+t7541-t7545+t7851+t2297.*(t5762-t6289-t6936+t6938+t7266-t7268)+t7846.*(t1861-t3214))+(t7.*t7978)./2.0+(t4.*t7983)./2.0-t4.*t7997+(t5.*t8003)./2.0-(t6.*t8004)./2.0-t5.*t8015-t7.*t8031;
et770 = (t2.*(-t6613-t6615+t7047+t7616+t6595.*(-t4007+t4011+t18.*(t1861-t3214).*1.838876e-2+t23.*(t1861-t3214).*9.99471e-3)))./2.0;
et771 = (t3.*(-t6614-t6616+t7047+t7616+t6595.*(-t4007+t4011+t18.*(t1861-t3214).*1.838876e-2+t23.*(t1861-t3214).*9.99471e-3)))./2.0;
et772 = t5338+t5340+t7725-t7727+t4149.*(t2674-t2676+t3022-t3027).*(t2694-t2701+t3036-t3043).*(t1488+t1874+t2519+t2740+t2747+t3096+t3097).*7.26735e-3+t4108.*(t2674-t2676+t3022-t3027).*(t2694-t2701+t3036-t3043).*(t1513+t1879+t2598+t2820+t2834+t3117+t3118).*7.26735e-3+t3877.*t3901.*t4149.*(t1488+t1874+t2519+t2740+t2747+t3096+t3097).*7.26735e-3;
et773 = t3877.*t3901.*t4108.*(t1513+t1879+t2598+t2820+t2834+t3117+t3118).*7.26735e-3;
et774 = -t2306-t2317+t3144+t3147+t35.*t941.*t948.*(t850-t874).*3.775747223193135e-1;
et775 = t36.*t941.*t948.*(t850-t874).*2.244797987218524e-1;
et776 = t50.*t189.*(-t4447+t4458+t3385.*(t2813-t2835+t18.*(t1456-t2355).*1.02e-6+t23.*(t1456-t2355).*9.0e-8)+t3386.*(-t2804+t2838+t3109+t23.*(t1456-t2355).*9.3e-7));
et777 = 9.543032792050485e-17;
et778 = t7484+(t5.*(-t6688-t6694+t6772+t6774+t7033+et776.*et777+t6561.*(t3547.*1.33637554986e-4+t4119-t4120+t34.*(t1896-t3232).*7.26350557185e-5)))./2.0-(t2.*t7631)./2.0-(t3.*t7632)./2.0-(t4.*t7745)./2.0;
et779 = (t6.*t7834)./2.0;
et780 = t50.*t189.*(-t4447+t4458+t3385.*(t2813-t2835+t18.*(t1456-t2355).*1.02e-6+t23.*(t1456-t2355).*9.0e-8)+t3386.*(-t2804+t2838+t3109+t23.*(t1456-t2355).*9.3e-7));
et781 = 9.543032792050485e-17;
et782 = t7484+(t5.*(-t6690-t6699+t6772+t6774+t7033+et780.*et781+t6561.*(t3547.*1.33637554986e-4+t4119-t4120+t34.*(t1896-t3232).*7.26350557185e-5)))./2.0-(t2.*t7633)./2.0-(t3.*t7635)./2.0-(t4.*t7746)./2.0;
et783 = (t6.*t7835)./2.0;
mt1 = [et398+et399,et433+et434+et435+et436,et589+et590+et591+et592,t5.*(et625+et626)-t2.*(et635+et636)+t6.*(et643+et644)-t3.*(et656+et657)+t4.*(et674+et675+et676)+t7.*(et677+et678+et679),-t3.*(t2.*t7785-(t2.*t7805)./2.0-(t3.*t7806)./2.0-(t4.*t7883)./2.0+(t6.*t7945)./2.0+(t7.*(et680+et681))./2.0+(t5.*(et686+et687))./2.0)+t4.*(et705+et706+et707)-t5.*(et714+et715)+t7.*(et720+et721+et722)+t2.*(t7749+(t2.*t7803)./2.0+(t3.*t7804)./2.0-(t6.*t7944)./2.0+(t5.*t7979)./2.0-(t4.*(et723+et724))./2.0)-t6.*(et754+et755+et756+et757)];
mt2 = [-t6.*(et762+et763+et764)+t7.*(et765+et766+et767+et768)-t5.*(et769+et770+et771)+t4.*(t4.*(et772+et773).*(-1.0./2.0)+t5.*(t7492-t7554+t7956+t7968-t7970+t7540.*(-t1901+t3122+t3270))+t4.*(t7570-t7973-t7974+t7540.*(et774+et775))-(t2.*t7796)./2.0-(t3.*t7797)./2.0+t2.*t7955+t3.*t7955+(t7.*t7985)./2.0-(t5.*t8001)./2.0-(t6.*t8002)./2.0+t6.*t8042+t7.*(t7498-t7568+t7959+t7975-t7977+t7540.*(t17.*((t237.*(t42-t43))./9.007199254740992e+15+t21.*(-t1881+t3121+t3269))+t22.*(-t1901+t3122+t3270))))-t2.*(et778+et779)-t3.*(et782+et783)];
tau_c = real(reshape([mt1,mt2],6,1));
end
